simulink library "thc"  (R2021b)
settings: Solver=VariableStepAuto  StartTime=0.0  StopTime=10.0  RelTol=1e-3
undefined symbols (not defined in the file): ATHC_APTCQA_X_C, ATHC_APTCQB_X_C, ATHC_dAy_X_C, ATHC_Qeq_X_kmh, ATHC_VbaseC_X_C, ATHC_VbaseC_Y_W, ATHC_VbaseD_X_C, ATHC_VbaseH_X_C, FALSE, KTHC_ACMaxMinT_sec, KTHC_aDeice_K, KTHC_AGSDefLv_K, KTHC_AGSLv1_K, KTHC_AGSLv2_K, KTHC_AGSLv3_K, KTHC_AGSLv4_K, KTHC_AGSLv5_K, KTHC_AirIntUpdateT_sec, KTHC_APTCOneZoneMax_W, KTHC_APTCPeriod_cnt, KTHC_APTCPWMEN_flg, KTHC_APTCQMaxC_W, KTHC_APTCQminC_W, KTHC_APTCQminD_W, KTHC_APTCQminRe1_W, KTHC_APTCQminRe_W, KTHC_APTCQoffT_cnt, KTHC_APTCQonT_cnt, KTHC_APTCRiLeMaxDff_W, KTHC_APTCRiLeMinDff_W, KTHC_BatCoolT_cnt, KTHC_BatInTempDef_C, KTHC_bDeice_K, KTHC_CompMaxDeice_rpm, KTHC_CompMinDeice_rpm, KTHC_CompSotxvOp_K, KTHC_CompSotxvOpLow_rpm, KTHC_CompSpdmax_rpm, KTHC_CompSpdmaxBC1_rpm, KTHC_CompSpdmaxBC_rpm, KTHC_CompSpdmid1_rpm, KTHC_CompSpdmid2_rpm, KTHC_CompSpdmid3_rpm, KTHC_CompSpdmid_rpm, KTHC_CompSpdmin_rpm, KTHC_DAPTCQ1_W, KTHC_DAPTCQ2_W, KTHC_DAPTCQ3_W, KTHC_DcChSetTemp_C, KTHC_DehumidityEN_flg, KTHC_DeiceCycTime_K, KTHC_DriveLevelWPTCBAH1_W, KTHC_DriveLevelWPTCBAH2_W, KTHC_DriveLevelWPTCBAH3_W, KTHC_DriveLevelWPTCBAH4_W, KTHC_DriverSeatPos_flg, KTHC_DriveT1MinBAH_C, KTHC_DriveT2MaxBAH_C, KTHC_DriveT2MinBAH_C, KTHC_DriveT3MaxBAH_C ... (+379)
libraries: simulink x489
(part 16 of 17)

== stateflow chart thc/THC/ThermalControl/THCM_Conctrl/Thermal ==
  state OFF
    en:CabinMode=0;CompPID=0;CompSet=0;SOTXV=false;BlowerPID=0;APTCPID=0;EXV2PIDMode=0;ACSubMode=0;
    BattPump3=0;FrWPTCHeatPwr=0;BatteryMode=0;EDriveMode=uint8(0);EWP1=0;EWP2=0;AGS=0;TWV=100;ACMaxReq=false;
    ACD3Lv=0;BattPump3=0;FAN=0;FWV=false;
  state ON
    state WaterFill
      en:CabinMode=1;
      CompPID=0;
      CompSet=0;
      SOTXV=false;
      BlowerPID=0;
      APTCPID=0;
      EXV2PIDMode=0;
      ACSubMode=0;
      FrWPTCHeatPwr=0;
      BatteryMode=0;
      EDriveMode=uint8(0);
      AGS=0;
      TWV=35;
      ACMaxReq=false;
      ACD3Lv=0;
      FAN=0;
      FWV=false;
      state WF1
        en:EWP1=7;
        EWP2=7;
        BattPump3=7;
      state WF2
        en:EWP1=0;
        EWP2=0;
        BattPump3=0;
      (default) -> (junction 2447)
      (junction 2447) -> (junction 2449) [order 2]
      (junction 2447) -> WF1 [order 1] : [WaterFillReq==1]
      (junction 2449) -> WF2
    state Normal
      state Cabin [parallel]
        settings: executionOrder=2
        state ForceSWMode [parallel]
          settings: executionOrder=8
          state StandBy
            en:CabinModeReset=false;
          state Cooling
            du:CabinModeReset=false;
          state Heating
            du:CabinModeReset=false;
          (default) -> ON.Normal.Cabin.ForceSWMode.StandBy
          ON.Normal.Cabin.ForceSWMode.Cooling -> ON.Normal.Cabin.ForceSWMode.Cooling [order 3] : [Tamb<sigSetTempZon1StC&&....
              | TambMax-Tamb>KTHC_ForceLeaveCool_C]
              | {CabinModeReset=true;TambMax=Tamb;}
          ON.Normal.Cabin.ForceSWMode.StandBy -> ON.Normal.Cabin.ForceSWMode.Cooling [order 1] : [CabinMode==3]{TambMax=Tamb;}
          ON.Normal.Cabin.ForceSWMode.Cooling -> ON.Normal.Cabin.ForceSWMode.StandBy [order 1] : [CabinMode!=3]
          ON.Normal.Cabin.ForceSWMode.Cooling -> ON.Normal.Cabin.ForceSWMode.Cooling [order 2] : [Tamb>TambMax]{TambMax=Tamb;}
          ON.Normal.Cabin.ForceSWMode.Heating -> ON.Normal.Cabin.ForceSWMode.Heating [order 2] : [TambMin>Tamb]{TambMin=Tamb;}
          ON.Normal.Cabin.ForceSWMode.StandBy -> ON.Normal.Cabin.ForceSWMode.Heating [order 2] : [CabinMode==8||CabinMode==9]
              | {TambMin=Tamb;}
          ON.Normal.Cabin.ForceSWMode.Heating -> ON.Normal.Cabin.ForceSWMode.Heating [order 3] : [Tamb>sigSetTempZon1St&&....
              | Tamb-TambMin>KTHC_ForceLeaveHeat_C]
              | {CabinModeReset=true;TambMin=Tamb;}
          ON.Normal.Cabin.ForceSWMode.Heating -> ON.Normal.Cabin.ForceSWMode.StandBy [order 1] : [CabinMode!=8&&CabinMode!=9]
        state CabinCompReqCtrl [parallel]
          settings: executionOrder=1
          state Request
            en:CabinCompReq=true;
            ForceComp=false;
            du:ForceComp=false;
          state NoRequest
            en:CabinCompReq=false;
            CabinCompReqCancel=false;
            du:CabinCompReqCancel=false;
          (default) -> ON.Normal.Cabin.CabinCompReqCtrl.Request
          ON.Normal.Cabin.CabinCompReqCtrl.Request -> ON.Normal.Cabin.CabinCompReqCtrl.NoRequest : [(CompSpd<=KTHC_CompSpdmin_rpm&&Tincar<sigSetTempZon1StC-KTHC_DTcabin5_C)||....
              | CabinCompReqCancel]
          ON.Normal.Cabin.CabinCompReqCtrl.NoRequest -> ON.Normal.Cabin.CabinCompReqCtrl.Request : [Tincar>sigSetTempZon1StC+KTHC_DTreturn_C||ForceComp]
        state Main [parallel]
          settings: executionOrder=2
          state DeiceMode
            en:CabinMode=10;CompPID=9;CompSet=0;SOTXV=true;EXV2PIDMode=0;
            ex:CompSet=0;
            state CompSet [parallel]
              settings: executionOrder=2
              CompSet -> (junction 2150) : {CompSet=Bat_Out_Temp*KTHC_aDeice_K+KTHC_bDeice_K;}
              (junction 2150) -> (junction 2152) [order 1] : [CompSet<KTHC_CompMinDeice_rpm]{CompSet=KTHC_CompMinDeice_rpm;}
              (junction 2150) -> (junction 2154) [order 2]
              (junction 2154) -> (junction 2156) [order 1] : [CompSet>KTHC_CompMaxDeice_rpm]{CompSet=KTHC_CompMaxDeice_rpm;}
              (junction 2154) -> (junction 2158) [order 2]
            state ModeSelect [parallel]
              settings: executionOrder=1
              state DeiceMode1
                en:ACSubMode=1;
                APTCPID=0;
                BlowerPID=0;
              state DeiceMode2
                en:ACSubMode=2;
                APTCPID=6;
                BlowerPID=4;
              (default) -> (junction 2045)
              (junction 2045) -> DeiceMode1 [order 1] : [!AC]
              (junction 2045) -> DeiceMode2 [order 2]
              DeiceMode1 -> DeiceMode2 : [AC]
              DeiceMode2 -> DeiceMode1 : [!AC]
          state ACStandbyMode
            state Mode1
              en:CabinMode=1;
              CompPID=0;CompSet=0;
              SOTXV=false;
              BlowerPID=0;
              APTCPID=0;
              EXV2PIDMode=0;
              ACSubMode=0;
            state Mode2
              en:CabinMode=2;SOTXV=true;SOTXV=true;
              BlowerPID=0;
              APTCPID=0;
              EXV2PIDMode=0;
              state ACStandByMode
                en:ACSubMode=1;
                CompPID=2;
                CompSet=0;
              state ACStandByMode2
                en:ACSubMode=2;
                CompPID=3;
                CompSet=KTHC_CompSpdmaxBC_rpm;
              (default) -> ACStandByMode
              ACStandByMode -> ACStandByMode2 : [TBMax>KTHC_TBPmax_C]
              ACStandByMode2 -> ACStandByMode : [TBMax<KTHC_TBPmin_C]
            (junction 733) -> (junction 740)
            (junction 740) -> ON.Normal.Cabin.Main.ACStandbyMode.Mode1 [order 1] : [RequestCOMP==0]
            (junction 740) -> (junction 753) [order 2]
            ON.Normal.Cabin.Main.ACStandbyMode.Mode2 -> ON.Normal.Cabin.Main.ACStandbyMode.Mode1 : [RequestCOMP==0]
            ON.Normal.Cabin.Main.ACStandbyMode.Mode1 -> ON.Normal.Cabin.Main.ACStandbyMode.Mode2 : [RequestCOMP==1]
            (junction 753) -> ON.Normal.Cabin.Main.ACStandbyMode.Mode2
          state DCCharge
            en:CabinMode=11;
            APTCPID=9;
            CompSet=0;
            EXV2PIDMode=0;
            BlowerPID=0;
            state CompOFF
              ACSubMode=2;
              CompPID=0;
              SOTXV=true;
            state CompON
              en:ACSubMode=1;
              CompPID=11;
              SOTXV=false;
            (default) -> (junction 2495)
            (junction 2495) -> ON.Normal.Cabin.Main.DCCharge.CompON [order 2]
            (junction 2495) -> ON.Normal.Cabin.Main.DCCharge.CompOFF [order 1] : [Bat_In_Temp>KTHC_TWinmax_C]
            ON.Normal.Cabin.Main.DCCharge.CompON -> ON.Normal.Cabin.Main.DCCharge.CompOFF : [Bat_In_Temp>KTHC_TWinmax_C]
            ON.Normal.Cabin.Main.DCCharge.CompOFF -> ON.Normal.Cabin.Main.DCCharge.CompON : [after(600,tick)&&Bat_In_Temp<KTHC_TWinmin_C]
          state ACON
            state Cooling
              en:CabinMode=3;
              EXV2PIDMode=0;
              state ACCooling
                en:APTCPID=5;
                state Normal
                  state ACCoolingMode1and7
                    en:
                    CompPID=1;
                    CompSet=0;
                    SOTXV=false;
                    state ACCoolingMode1
                      en:BlowerPID=1;
                      ACSubMode=1;
                    state ACCoolingMode0
                      en:BlowerPID=0;
                      ACSubMode=0;
                    (default) -> (junction 2391)
                    (junction 2391) -> (junction 2393) [order 2]
                    (junction 2391) -> ACCoolingMode1 [order 1] : [FCool==0]
                    (junction 2393) -> ACCoolingMode0
                    ACCoolingMode0 -> ACCoolingMode1 : [FCool==0]
                    ACCoolingMode1 -> ACCoolingMode0 : [FCool>0]
                  state ACCoolingMode1_2
                    ex:APTCPID=5;
                    state Dehumidity
                      en:CabinMode=6;
                      ACSubMode=2;
                      CompPID=3;
                      BlowerPID=1;
                      SOTXV=false;
                      CompSet=KTHC_CompSpdmid3_rpm;
                      APTCPID=7;
                      ex:CabinMode=3;
                    state CompON
                      en:CabinMode=3;
                      APTCPID=8;
                      CompSet=0;
                      state ACCoolingMode6
                        en:
                        ACSubMode=6;
                        CompPID=10;
                        BlowerPID=0;
                        SOTXV=false;
                      state ACCoolingMode7
                        en:
                        ACSubMode=7;
                        CompPID=3;
                        BlowerPID=0;
                        SOTXV=true;
                      state ACCoolingMode2
                        en:
                        ACSubMode=2;
                        CompPID=10;
                        BlowerPID=1;
                        SOTXV=false;
                      (default) -> (junction 2413)
                      ON.Normal.Cabin.Main.ACON.Cooling.ACCooling.Normal.ACCoolingMode1_2.CompON -> (junction 2413) [order 1] : [hasChanged(FCool)]
                      (junction 2413) -> (junction 2420) [order 2]
                      (junction 2420) -> (junction 2431) [order 2]
                      (junction 2413) -> ACCoolingMode2 [order 1] : [FCool==0]
                      (junction 2420) -> ACCoolingMode6 [order 1] : [FCool==1]
                      (junction 2431) -> ACCoolingMode7
                    (default) -> (junction 2498)
                    (junction 2498) -> ON.Normal.Cabin.Main.ACON.Cooling.ACCooling.Normal.ACCoolingMode1_2.CompON [order 2]
                    (junction 2498) -> Dehumidity [order 1] : [Tincar<sigSetTempZon1StC-KTHC_DTcabin2_C&&....
                        | sigSetTempZon1St>17&&....
                        | (Tamb<KTHC_TambACmode7_C||....
                        | sigSetTempZon1StC>Tamb+KTHC_DTambsat4_C)]
                    Dehumidity -> ON.Normal.Cabin.Main.ACON.Cooling.ACCooling.Normal.ACCoolingMode1_2.CompON [order 2] : [(after(KTHC_DTimeCD1_K,tick)&&....
                        | Tincar>sigSetTempZon1StC+KTHC_DTcabin1_C)&&....
                        | (Tamb>KTHC_TambACmode6_C||....
                        | sigSetTempZon1StC<Tamb-KTHC_DTambsat3_C)||....
                        | sigSetTempZon1St<=17]
                    ON.Normal.Cabin.Main.ACON.Cooling.ACCooling.Normal.ACCoolingMode1_2.CompON -> Dehumidity [order 1] : [Tincar<sigSetTempZon1StC-KTHC_DTcabin2_C&&....
                        | sigSetTempZon1St>17&&....
                        | (Tamb<KTHC_TambACmode7_C||....
                        | sigSetTempZon1StC>Tamb+KTHC_DTambsat4_C)]
                  state ACCoolingMode1_3
                    en:ACSubMode=3;
                    CompPID=2;
                    CompSet=0;
                    BlowerPID=1;
                    SOTXV=!TincarPos;
                    du:SOTXV=!TincarPos;
                  ACCoolingMode1_2 -> ACCoolingMode1and7 [order 2] : [CabinCompReq]
                  (default) -> (junction 2360)
                  (junction 2360) -> ACCoolingMode1and7 [order 1] : [ACSubModeLAST == 1]
                  (junction 2360) -> ACCoolingMode1_2 [order 2] : [ACSubModeLAST == 2]
                  (junction 2360) -> (junction 2364) [order 3]
                  (junction 777) -> ACCoolingMode1_2 [order 1] : [RequestCOMP==0]
                  ACCoolingMode1_2 -> ACCoolingMode1_3 [order 1] : [RequestCOMP]
                  ACCoolingMode1_3 -> ACCoolingMode1_2 [order 2] : [!RequestCOMP]
                  ACCoolingMode1and7 -> (junction 777) [order 3] : [!CabinCompReq]
                  (junction 777) -> ACCoolingMode1_3 [order 2]
                  (junction 2364) -> ACCoolingMode1_3
                  ACCoolingMode1and7 -> ACCoolingMode1_3 [order 2] : [WaterCompReq]
                  ACCoolingMode1_3 -> ACCoolingMode1and7 [order 1] : [CabinCompReq&&....
                      | !WaterCompReq]
                state ACCoolingMode1_4
                  en:ACSubMode=4;CompPID=0;
                  CompSet=KTHC_CompSpdmaxBC1_rpm;BlowerPID=1;
                  SOTXV=!TincarPos;
                  du:SOTXV=!TincarPos;
                ACCoolingMode1_4 -> ACCoolingMode1_3 : [TBMax<KTHC_TBPmin_C]
                (junction 2357) -> ON.Normal.Cabin.Main.ACON.Cooling.ACCooling.Normal [order 2]
                ON.Normal.Cabin.Main.ACON.Cooling.ACCooling.Normal -> ACCoolingMode1_4 : [TBMax>KTHC_TBPmax_C]
                (junction 2357) -> ACCoolingMode1_4 [order 1] : [ACSubModeLAST == 4]
              state ACCoolingMode1_5
                en:
                BlowerPID=1;
                SOTXV=true;
                APTCPID=0;
                state CompMax
                  en:
                  CompPID=0;
                  CompSet=KTHC_CompSpdmaxBC1_rpm;
                state CompWin
                  en:
                  CompPID=2;
                  CompSet=0;
                state CompOFF
                  en:
                  CompPID=0;
                  CompSet=0;
                (junction 1698) -> (junction 1701) [order 2] : {ACSubMode=5;}
                (junction 1701) -> (junction 1705) [order 2]
                (junction 1698) -> CompMax [order 1] : [ACSubMode==4]{ACSubMode=5;}
                (junction 1701) -> CompWin [order 1] : [RequestCOMP]
                (junction 1705) -> ON.Normal.Cabin.Main.ACON.Cooling.ACCoolingMode1_5.CompOFF
                CompWin -> CompMax [order 1] : [TBMax>KTHC_TBPmax_C]
                CompWin -> ON.Normal.Cabin.Main.ACON.Cooling.ACCoolingMode1_5.CompOFF [order 2] : [!RequestCOMP]
                ON.Normal.Cabin.Main.ACON.Cooling.ACCoolingMode1_5.CompOFF -> CompWin : [RequestCOMP]
                CompMax -> CompWin : [TBMax<KTHC_TBPmin_C]
              (default) -> ACCoolingMode1and7
              ACCoolingMode1_5 -> (junction 2357) : [!EvapDefog]
              ACCooling -> (junction 1698) : [EvapDefog&&....
                  | Tamb>=KTHC_Trecymin_C]{ACSubModeLAST = ACSubMode;}
            state Duhumidity
              state DehumidityMode1and2
                state DehumidityMode1
                  en:CabinMode=4;ACSubMode=0;
                  CompPID=6;BlowerPID=3;
                  EXV2PIDMode=0;
                  APTCPID=5;SOTXV=false;
                state DehumidityMode2
                  en:CabinMode=5;
                  BlowerPID=3;
                  EXV2PIDMode=2;
                  SOTXV=false;
                  state DehumidityMode21
                    en:ACSubMode=1;
                    APTCPID=5;
                    CompPID=6;
                  state DehumidityMode22
                    en:ACSubMode=2;
                    APTCPID=2;
                    CompPID=8;
                  (default) -> DehumidityMode21
                  DehumidityMode21 -> DehumidityMode22 [order 1] : [after(100,tick)&&....
                      | (CompSpd>=KTHC_CompSpdmax_rpm||....
                      | ACHP>=KTHC_PhiDehum_kPa||....
                      | PT_High_T>=KTHC_ThiDehum_C)]
                  DehumidityMode22 -> DehumidityMode21 : [(after(KTHC_TimeD_K,tick)||....
                      | Tincar>sigSetTempZon1St+1)&&....
                      | APTCQ<=APTCQminD]
                DehumidityMode1and2 -> DehumidityMode22 [order 1] : [ErrCompForceOFF]
                (junction 1764) -> DehumidityMode1 [order 1] : [Tamb>KTHC_TambACmode2_C]
                (junction 1764) -> DehumidityMode2 [order 2] : [Tamb>KTHC_TambACmode3_C]
                DehumidityMode21 -> DehumidityMode1 [order 2] : [(CompSpd<=KTHC_CompSpdmin_rpm&&....
                    | Tincar>sigSetTempZon1St+KTHC_DTcabin3_C)||....
                    | (after(100,tick)&&....
                    | CompSpd<=KTHC_CompSpdmid1_rpm&&....
                    | Tincar>sigSetTempZon1St+KTHC_DTcabin12_C)]
                DehumidityMode1 -> DehumidityMode2 [order 2] : [CompSpd>KTHC_CompSpdmid_rpm||....
                    | ACHP>=KTHC_PhiDehum_kPa||....
                    | PT_High_T>KTHC_ThiDehum_C]
              state DehumidityMode4
                en:CabinMode=7;
                ACSubMode=0;
                CompPID=7;
                BlowerPID=3;
                EXV2PIDMode=0;
                SOTXV=true;
                APTCPID=4;
              state DehumidityMode3
                en:CabinMode=6;
                ACSubMode=1;
                CompPID=7;
                BlowerPID=3;
                EXV2PIDMode=0;
                SOTXV=false;
                APTCPID=3;
                FanMax=false;
                ex:ACD3Lv=0;
                state L2
                  en:ACD3Lv=2;
                state L3
                  en:ACD3Lv=3;
                state L4
                  en:ACD3Lv=4;
                state L5
                  en:ACD3Lv=5;
                  state Wait
                  state MAX
                    en:FanMax=true;
                  (default) -> ON.Normal.Cabin.Main.ACON.Duhumidity.DehumidityMode3.L5.Wait
                  ON.Normal.Cabin.Main.ACON.Duhumidity.DehumidityMode3.L5.Wait -> MAX : [after(150,tick)]
                (default) -> L2
                (junction 1803) -> L2 [order 1] : [Tincar<sigSetTempZon1St-1]
                L2 -> L3 : [Tincar>sigSetTempZon1St+1]
                L3 -> (junction 1803) : [after(150,tick)]
                (junction 1803) -> L4 [order 2] : [Tincar>sigSetTempZon1St+1]
                (junction 1808) -> L3 [order 1] : [Tincar<sigSetTempZon1St-1]
                L4 -> (junction 1808) : [after(150,tick)]
                (junction 1808) -> L5 [order 2] : [Tincar>sigSetTempZon1St+1]
                L5 -> L4 : [Tincar<sigSetTempZon1St-1]....
                    | {FanMax=false;}
              DehumidityMode3 -> DehumidityMode21 [order 1] : [!RequestCOMP]
              DehumidityMode1and2 -> DehumidityMode3 [order 3] : [RequestCOMP]
              DehumidityMode3 -> DehumidityMode4 [order 2] : [EvapDefog]
              DehumidityMode4 -> DehumidityMode3 [order 2] : [!EvapDefog]
            state HeatingMode
              en:ReqWasteHeatRecovery=true;SOTXV=true;
              ex:ReqWasteHeatRecovery=false;
              state HeatingMode1
                en:CabinMode=8;
                state HeatingMode11
                  en:CompPID=4;
                  APTCPID=5;
                  EXV2PIDMode=1;
                  ACSubMode=1;
                  BlowerPID=2;
                state HeatingMode12
                  en:CompPID=3;
                  APTCPID=5;
                  ACSubMode=2;
                  BlowerPID=2;
                  state EXV2ON
                    en:
                    EXV2PIDMode=1;
                    CompSet=KTHC_CompSpdmin_rpm;
                  state EXV2OFF
                    en:
                    EXV2PIDMode=0;
                    CompSet=0;
                  (default) -> EXV2ON
                  EXV2OFF -> EXV2ON : [Tincar<sigSetTempZon1St-KTHC_DTcabin9_C]
                  EXV2ON -> EXV2OFF : [Tincar>sigSetTempZon1St+KTHC_DTcabin9_C]
                HeatingMode11 -> HeatingMode12 [order 4] : [CompSpd<=KTHC_CompSpdmin_rpm&&....
                    | Tincar>sigSetTempZon1St+KTHC_DTcabin10_C]
                HeatingMode12 -> HeatingMode11 : [Tincar<sigSetTempZon1St-KTHC_DTreturn6_C]
              state HeatingMode2
                en:CabinMode=9;
                state HeatingMode21
                  en:CompPID=5;
                  APTCPID=1;
                  EXV2PIDMode=1;
                  ACSubMode=1;
                  BlowerPID=2;
                state APTCStart
                  en:CompPID=5;
                  APTCPID=1;
                  EXV2PIDMode=1;
                  BlowerPID=2;
                  ACSubMode=1;
                  state APTCStart
                  state APTCWait
                  (default) -> ON.Normal.Cabin.Main.ACON.HeatingMode.HeatingMode2.APTCStart.APTCStart
                  APTCWait -> ON.Normal.Cabin.Main.ACON.HeatingMode.HeatingMode2.APTCStart.APTCStart [order 1] : [APTCQ>KTHC_APTCQminRe1_W]
                  ON.Normal.Cabin.Main.ACON.HeatingMode.HeatingMode2.APTCStart.APTCStart -> APTCWait : [(!DfrstReq||Tincar>sigSetTempZon1St+KTHC_DTCabin11_C)&&....
                      | APTCQ<KTHC_APTCQminRe_W]{ACMaxReq=false;}
                state HeatingMode22
                  en:CompPID=0;
                  APTCPID=1;
                  EXV2PIDMode=0;
                  ACSubMode=2;
                  BlowerPID=2;
                  CompSet=0;
                HeatingMode21 -> ON.Normal.Cabin.Main.ACON.HeatingMode.HeatingMode2.APTCStart [order 1] : [APTCQ>=KTHC_APTCQminRe_W]
                ON.Normal.Cabin.Main.ACON.HeatingMode.HeatingMode2.APTCStart -> HeatingMode22 : [(EACProtectEnable==1||....
                    | PT_Low_P2<=KTHC_Plow2Setpoint_kPa)&&....
                    | CompSpd<=KTHC_CompSpdmin_rpm]
                (junction 2279) -> ON.Normal.Cabin.Main.ACON.HeatingMode.HeatingMode2.APTCStart : [(Motor_Out_Temp>KTHC_Twmset_C&&....
                    | PT_Low_P2>KTHC_Plow2Setpoint_kPa)||....
                    | Tamb>KTHC_Tambset_C]
                HeatingMode22 -> (junction 2279) : [after(3000,tick)]
              (default) -> (junction 972)
              (junction 972) -> (junction 973) [order 2]
              (junction 973) -> HeatingMode21
              (junction 972) -> HeatingMode11 [order 1] : [Tamb>KTHC_TambACmode4_C]
              HeatingMode11 -> HeatingMode21 [order 1] : [after(Timehu1,tick)&&Tincar<KTHC_DTh1_C]
              HeatingMode11 -> HeatingMode21 [order 2] : [after(Timehu2,tick)&&....
                  | (EACProtectEnable==1||CompSpd>=KTHC_CompSpdmax_rpm)&&Tincar<sigSetTempZon1St-KTHC_DTCabin11_C]
              HeatingMode11 -> HeatingMode21 [order 3] : [ACMaxReq||(DfrstReq&&Tincar<sigSetTempZon1St-KTHC_DTCabin11_C)]
              HeatingMode21 -> HeatingMode11 [order 2] : [after(KTHC_TimeRe2_sec*10,tick)&&Tincar>sigSetTempZon1St+KTHC_DTCabin11_C]
              APTCWait -> HeatingMode11 [order 2] : [after(KTHC_TimeRe1_sec*10,tick)]
            (junction 759) -> (junction 729)
            (junction 729) -> (junction 2287) [order 2]
            (junction 2287) -> (junction 724) [order 2]
            (junction 724) -> (junction 739) [order 2]
            (junction 729) -> ACCoolingMode1and7 [order 1] : [(!Tamb_Err&&(Tamb>KTHC_TambACmode1_C||(Tamb>KTHC_TambACmode3_C&&!KTHC_DehumidityEN_flg)))||(Tamb_Err&&Tincar>=sigSetTempZon1St)]
            (junction 2287) -> DehumidityMode1 [order 1] : [Tamb_Err]
            (junction 724) -> (junction 1764) [order 1] : [KTHC_DehumidityEN_flg]
            (junction 739) -> HeatingMode
            DehumidityMode1and2 -> ACCoolingMode1and7 [order 2] : [(!RequestCOMP&&Tincar>sigSetTempZon1StC+KTHC_DTcabin7_C&&....
                | sigSetTempZon1StC<Tamb-KTHC_DTambSat2_C)||....
                | Tincar>sigSetTempZon1StC+KTHC_DTreturn7_C||....
                | sigSetTempZon1St<=17]{ForceComp=true;}
            ACCoolingMode1and7 -> DehumidityMode1 [order 1] : [Tincar<sigSetTempZon1StC-KTHC_DTreturn1_C&&....
                | sigSetTempZon1StC>Tamb+KTHC_DTambSat1_C&&....
                | sigSetTempZon1St>17]
            DehumidityMode1 -> Dehumidity [order 1] : [(!RequestCOMP&&CompSpd<=KTHC_CompSpdmid2_rpm&&....
                | Tincar>sigSetTempZon1StC+KTHC_DTcabin4_C&&....
                | Tamb>KTHC_TambACmode5_C&&....
                | after(KTHC_DTimeCD2_K,tick))||....
                | (CompSpd<=KTHC_CompSpdmin_rpm&&....
                | ACHP>=KTHC_PhiDehum_kPa)]{CabinCompReqCancel=true;}...
            Dehumidity -> DehumidityMode1 [order 1] : [after(KTHC_DTimeCD_K,tick)&&...
                | KTHC_DehumidityEN_flg&&....
                | (Tincar<sigSetTempZon1StC-KTHC_DTreturn3_C||....
                | APTCQ>KTHC_APTCQMaxC_W)&&....
                | Tamb-sigSetTempZon1StC<KTHC_DTambSat_C]
            HeatingMode -> DehumidityMode22 [order 2] : [KTHC_DehumidityEN_flg&&...
                | !EvapDefog&&....
                | Tamb>KTHC_Tdeheat2_C]
            DehumidityMode1and2 -> HeatingMode21 [order 1] : [EvapDefog||Tamb<KTHC_Tdeheat1_C]
            DehumidityMode4 -> HeatingMode21 [order 1] : [!RequestCOMP]
            HeatingMode -> DehumidityMode4 [order 1] : [KTHC_DehumidityEN_flg&&RequestCOMP]
            DehumidityMode3 -> ACCoolingMode1_3 [order 3] : [FanMax&&Tincar>sigSetTempZon1St+KTHC_DTcabin6_C]
            ACCoolingMode1_3 -> DehumidityMode3 [order 3] : [KTHC_DehumidityEN_flg&&....
                | Tincar<sigSetTempZon1StC-KTHC_DTreturn2_C&&....
                | Tamb-sigSetTempZon1StC<KTHC_DTambSat_C]
            HeatingMode -> ON.Normal.Cabin.Main.ACON.Cooling [order 3] : [!KTHC_DehumidityEN_flg&&Tamb>=sigSetTempZon1St||....
                | (sigSetTempZon1St<=17&&Tamb>KTHC_TambSetLow_C)]
            ON.Normal.Cabin.Main.ACON.Cooling -> HeatingMode : [!KTHC_DehumidityEN_flg&&Tamb<sigSetTempZon1St]
          (default) -> (junction 761)
          (junction 761) -> (junction 733) [order 2]
          ACStandbyMode -> DeiceMode [order 2] : [DeiceModeReq==1]
          (junction 761) -> (junction 759) [order 1] : [(PwrSta>3&&AC)||....
              | (PwrSta>0&&PET)]
          ACON -> (junction 733) [order 2] : [(PwrSta<=3||!AC)&&....
              | (!PET||PwrSta==0)]
          (junction 2484) -> ON.Normal.Cabin.Main.ACStandbyMode.Mode1
          (junction 1972) -> (junction 2484) [order 2]
          DeiceMode -> (junction 1972) : [DeiceModeReq==0]
          ON.Normal.Cabin.Main.DCCharge -> (junction 2484) : [BatteryMode!=7]
          (junction 1972) -> (junction 973) [order 1] : [AC]
          ACON -> DeiceMode [order 3] : [DeiceModeReq==1]
          ACStandbyMode -> ON.Normal.Cabin.Main.DCCharge [order 3] : [BatteryMode==7]
          ACON -> ON.Normal.Cabin.Main.DCCharge [order 1] : [BatteryMode==7]
          ACStandbyMode -> (junction 729) [order 1] : [(PwrSta>3&&AC)||....
              | (PwrSta>0&&PET)]
          Main -> (junction 759) : [CabinModeReset]
        state WaterCompReqCtrl [parallel]
          settings: executionOrder=3
          state CoolingON
            note: 15 min
            state Request
              en:WaterCompReq=true;
            state ON
            state NoRequest
              en:WaterCompReq=false;
            ON.Normal.Cabin.WaterCompReqCtrl.CoolingON.ON -> (junction 1745) : [after(KTHC_Timewcd_K,tick)]
            (junction 1745) -> ON.Normal.Cabin.WaterCompReqCtrl.CoolingON.Request [order 1] : [RequestCOMP==1&&....
                | TBMax>=KTHC_T3MaxBC_C&&....
                | Bat_In_Temp>KTHC_T3winSetpointBC_C]....
            (junction 1745) -> (junction 1748) [order 2]
            ON.Normal.Cabin.WaterCompReqCtrl.CoolingON.Request -> ON.Normal.Cabin.WaterCompReqCtrl.CoolingON.NoRequest : [RequestCOMP==0||....
                | TBMax<KTHC_T4MinBC_C]
            ON.Normal.Cabin.WaterCompReqCtrl.CoolingON.NoRequest -> ON.Normal.Cabin.WaterCompReqCtrl.CoolingON.Request : [RequestCOMP==1&&....
                | TBMax>=KTHC_T3MaxBC_C&&....
                | Bat_In_Temp>KTHC_T3winSetpointBC_C]....
            (junction 1748) -> ON.Normal.Cabin.WaterCompReqCtrl.CoolingON.NoRequest
          state OFF
            en:WaterCompReq=false;
          (default) -> ON.Normal.Cabin.WaterCompReqCtrl.OFF
          ON.Normal.Cabin.WaterCompReqCtrl.OFF -> ON.Normal.Cabin.WaterCompReqCtrl.CoolingON.ON : [CabinMode==3]
          CoolingON -> ON.Normal.Cabin.WaterCompReqCtrl.OFF : [CabinMode!=3]
        state EvapDefogCtrl [parallel]
          settings: executionOrder=4
          state OFF
            en:EvapDefog=false;
          state ON
            en:EvapDefog=true;
          (default) -> ON.Normal.Cabin.EvapDefogCtrl.OFF
          ON.Normal.Cabin.EvapDefogCtrl.OFF -> ON.Normal.Cabin.EvapDefogCtrl.ON : [Tevap<Tice]
          ON.Normal.Cabin.EvapDefogCtrl.ON -> ON.Normal.Cabin.EvapDefogCtrl.OFF : [Tevap>Tdeice]
        state ACMaxReq [parallel]
          settings: executionOrder=6
          state OFF
            en:ACMaxReq=false;
          state ON
            en:ACMaxReq=true;
          (default) -> ON.Normal.Cabin.ACMaxReq.OFF
          ON.Normal.Cabin.ACMaxReq.OFF -> ON.Normal.Cabin.ACMaxReq.ON : [ACMax]
          ON.Normal.Cabin.ACMaxReq.ON -> ON.Normal.Cabin.ACMaxReq.OFF : [!ACMax]
        state ForceCool [parallel]
          settings: executionOrder=7
          state Normal
            en:FCool=0;
          state ForceCool
            state ForceCool2
              en:FCool=2;
            state ForceCool1
              en:FCool=1;
            (junction 2403) -> (junction 2408) [order 2] : [Tamb<KTHC_Trecymin_C]
            (junction 2403) -> ForceCool1 [order 1] : [Tamb>=KTHC_Trecymin_C]
            (junction 2408) -> ForceCool2
            ForceCool1 -> ForceCool2 : [Tamb<KTHC_Trecymin_C]
            ForceCool2 -> ForceCool1 : [Tamb>=KTHC_Trecymin_C]
          (default) -> ON.Normal.Cabin.ForceCool.Normal
          ON.Normal.Cabin.ForceCool.Normal -> (junction 2403) : [sigSetTempZon1St<=17&&....
              | Tamb<KTHC_Tcoolmin_C]
          ON.Normal.Cabin.ForceCool.ForceCool -> ON.Normal.Cabin.ForceCool.Normal : [sigSetTempZon1St>17||....
              | Tamb>=KTHC_Tcoolmin_C]
        state TincarPos [parallel]
          settings: executionOrder=5
          state Up
            TincarPos=true;
          state Down
            TincarPos=false;
          (default) -> (junction 1725)
          (junction 1725) -> Up [order 1] : [Tincar>sigSetTempZon1StC+KTHC_DTcabin_C]
          (junction 1725) -> (junction 1717) [order 2]
          Up -> Down : [Tincar<sigSetTempZon1StC-KTHC_DTcabin_C]
          Down -> Up : [Tincar>sigSetTempZon1StC+KTHC_DTcabin_C]
          (junction 1717) -> Down
      state Battery [parallel]
        settings: executionOrder=3
        state Battery [parallel]
          settings: executionOrder=3
          state Normal
            state Mode1
              en:BatteryMode=1;
              RequestCOMP=1;
              ex:RequestCOMP=0;
            state Mode2
              en:BatteryMode=2;
              FWV=true;
              ex:FWV=false;
            state Mode3
              en:BatteryMode=3;
            state Mode4
              en:BatteryMode=4;
              RequestTWV=1
              FWV=true;
              ex:RequestTWV=0;
              FWV=false;
            state Mode5
              en:BatteryMode=5;
            (default) -> (junction 600)
            (junction 600) -> ON.Normal.Battery.Battery.Normal.Mode1 [order 1] : [TBMax>KTHC_T1MaxBC_C]
            (junction 600) -> (junction 603) [order 2]
            ON.Normal.Battery.Battery.Normal.Mode1 -> ON.Normal.Battery.Battery.Normal.Mode2 [order 1] : [after(1200,tick)&&....
                | TBMin-Motor_In_Temp>KTHC_DTwBMoin1_C&&....
                | TBMax<KTHC_T4MinBC_C-1&&....
                | ChrgPlugSta<2]
            ON.Normal.Battery.Battery.Normal.Mode2 -> ON.Normal.Battery.Battery.Normal.Mode1 [order 2] : [TBMax>KTHC_T3MaxBC_C||....
                | (TBMin-Bat_In_Temp<KTHC_DTwBBin_C&&....
                | after(1200,tick))]
            (junction 601) -> ON.Normal.Battery.Battery.Normal.Mode1 [order 2]
            Mode3 -> ON.Normal.Battery.Battery.Normal.Mode1 [order 3] : [ChrgPlugSta==2&&....
                | TBMax>KTHC_TDcChgBC_C]
            ON.Normal.Battery.Battery.Normal.Mode1 -> Mode3 [order 2] : [(TBMax<KTHC_T2MinBC_C&&....
                | ChrgPlugSta<2)||....
                | (TBMax<KTHC_TDcChgBC_C-2&&....
                | ChrgPlugSta==2)]
            (junction 601) -> ON.Normal.Battery.Battery.Normal.Mode2 [order 1] : [TBMin-Motor_In_Temp>KTHC_DTwBMoin1_C]
            Mode3 -> (junction 601) [order 1] : [TBMax>KTHC_T1MaxBC_C&&....
                | ChrgPlugSta<2]
            ON.Normal.Battery.Battery.Normal.Mode2 -> Mode3 [order 1] : [TBMax<KTHC_T2MinBC_C]
            (junction 603) -> Mode3 [order 1] : [TBMin>=KTHC_T1MinBH_C]
            (junction 603) -> (junction 606) [order 2]
            Mode4 -> Mode3 [order 1] : [TBMin>KTHC_T2MaxBH_C||....
                | (ChrgPlugSta==0&&....
                | PreWPTC==0&&....
                | after(1200,tick)&&....
                | Bat_In_Temp-TBMax<=0&&....
                | TBMin>=KTHC_T2MinBH_C)]
            Mode3 -> (junction 604) [order 2] : [TBMin<KTHC_T1MinBH_C]
            Mode5 -> Mode3 [order 1] : [TBMin>KTHC_T2MaxBH_C||....
                | (ChrgPlugSta==0&&....
                | PreWPTC==0&&....
                | TBMin>=KTHC_T3MaxBH_C&&...
                | Motor_In_Temp-TBMax<=0)]
            (junction 604) -> Mode4 [order 2] : [Motor_In_Temp-TBMax>KTHC_DTwBMoin2_C]
            (junction 604) -> Mode5 [order 1] : [ChrgPlugSta>0||....
                | PreWPTC==1||....
                | TBMin<KTHC_T2MinBH_C]
            Mode4 -> Mode5 [order 2] : [((ChrgPlugSta>0||....
                | PreWPTC==1)&&....
                | TBMin<=KTHC_T2MaxBH_C)||....
                | (after(1200,tick)&&....
                | TBMin<KTHC_T2MinBH_C)]
            Mode5 -> Mode4 [order 2] : [ChrgPlugSta==0&&....
                | PreWPTC==0&&....
                | TBMin>=KTHC_T3MaxBH_C&&....
                | Motor_In_Temp-TBMax>KTHC_DTwBMoin3_C]
            (junction 606) -> Mode5
          state Deicing
            en:BatteryMode=6;
          note: BatteryMode
              | 0=OFF;
              | 1=Active Cooling;
              | 2=Passing Cooling;
              | 3=Isothermal Cycle;
              | 4=Passive Heating;
              | 5=Active Heating;
              | 6=Deicing;
          state BatteryDCChargeHeatingWoWPTC
            en:BatteryMode=7;
            BatDcCharge=true;
            ex:BatDcCharge=false;
            state Wait
            state FWVON
              en:FWV=true;
              ex:FWV=false;
            (default) -> ON.Normal.Battery.Battery.BatteryDCChargeHeatingWoWPTC.Wait
            ON.Normal.Battery.Battery.BatteryDCChargeHeatingWoWPTC.Wait -> FWVON : [after(50,tick)]
          state WaitForBalance
          (default) -> ON.Normal.Battery.Battery.Normal
          ON.Normal.Battery.Battery.Deicing -> (history) : [DeiceModeReq==0]
          ON.Normal.Battery.Battery.Normal -> ON.Normal.Battery.Battery.Deicing : [DeiceModeReq]
          WaitForBalance -> Mode3 : [after(50,tick)]
          BatteryDCChargeHeatingWoWPTC -> WaitForBalance : [!KTHC_WoWPTC_flg||....
              |  ChrgPlugSta!=2||....
              | TBMin>KTHC_T2MaxBH_C]
          Mode5 -> BatteryDCChargeHeatingWoWPTC [order 3] : [KTHC_WoWPTC_flg && ChrgPlugSta==2]
        state BattPump3 [parallel]
          settings: executionOrder=4
          state ON
            state OFF
              en:
              BattPump3=0;
              PumpONmode = 0;
            state Cooling
              en:
              PumpONmode = 1;
              state Level2
                en:BattPump3=2;
              state Level3
                en:BattPump3=3;
              state Level4
                en:BattPump3=4;
              state Level5
                en:BattPump3=5;
              (default) -> (junction 1568)
              (junction 1568) -> ON.Normal.Battery.BattPump3.ON.Cooling.Level2 [order 1] : [BattPump3<=2]
              (junction 1568) -> (junction 1570) [order 2]
              ON.Normal.Battery.BattPump3.ON.Cooling.Level2 -> ON.Normal.Battery.BattPump3.ON.Cooling.Level3 : [TBMax>KTHC_T2MaxBC_C]
              ON.Normal.Battery.BattPump3.ON.Cooling.Level3 -> ON.Normal.Battery.BattPump3.ON.Cooling.Level2 [order 2] : [TBMax<KTHC_T3MinBC_C]
              (junction 1570) -> ON.Normal.Battery.BattPump3.ON.Cooling.Level3 [order 1] : [BattPump3==3]
              (junction 1570) -> (junction 1573) [order 2]
              ON.Normal.Battery.BattPump3.ON.Cooling.Level3 -> ON.Normal.Battery.BattPump3.ON.Cooling.Level4 [order 1] : [TBMax>KTHC_T3MaxBC_C]
              ON.Normal.Battery.BattPump3.ON.Cooling.Level4 -> ON.Normal.Battery.BattPump3.ON.Cooling.Level3 [order 1] : [TBMax<KTHC_T4MinBC_C]
              (junction 1573) -> ON.Normal.Battery.BattPump3.ON.Cooling.Level4 [order 1] : [BattPump3==4]
              (junction 1573) -> (junction 1576) [order 2]
              ON.Normal.Battery.BattPump3.ON.Cooling.Level4 -> ON.Normal.Battery.BattPump3.ON.Cooling.Level5 [order 2] : [TBMax>KTHC_T4MaxBC_C]
              ON.Normal.Battery.BattPump3.ON.Cooling.Level5 -> ON.Normal.Battery.BattPump3.ON.Cooling.Level4 : [TBMax<KTHC_T5MinBC_C]
              (junction 1576) -> ON.Normal.Battery.BattPump3.ON.Cooling.Level5
            state IsothermalCycle
              en:
              PumpONmode = 2;
              state Level2
                en:BattPump3=1;
                state Higher3
                state Lower3
                (default) -> Higher3
                Lower3 -> Higher3 [order 1] : [TBMax-TBMin>3]
                Higher3 -> Lower3 : [TBMax-TBMin<=3]
              state Level4
                en:BattPump3=4;
              state Level3
                en:BattPump3=3;
              note: 5 min
              state Level1
                en:BattPump3=0;
              (default) -> (junction 674)
              (junction 673) -> (junction 674)
              (junction 674) -> (junction 675) [order 2]
              (junction 675) -> (junction 676) [order 2]
              (junction 676) -> (junction 2585) [order 1] : [TBMax-TBMin<2]
              (junction 677) -> (junction 673)
              (junction 674) -> ON.Normal.Battery.BattPump3.ON.IsothermalCycle.Level4 [order 1] : [TBMax-TBMin>=7]
              (junction 675) -> ON.Normal.Battery.BattPump3.ON.IsothermalCycle.Level3 [order 1] : [TBMax-TBMin>=5]
              (junction 676) -> ON.Normal.Battery.BattPump3.ON.IsothermalCycle.Level2 [order 2]
              (junction 2585) -> ON.Normal.Battery.BattPump3.ON.IsothermalCycle.Level1
              ON.Normal.Battery.BattPump3.ON.IsothermalCycle.Level4 -> (junction 678) : [TBMax-TBMin<7]
              ON.Normal.Battery.BattPump3.ON.IsothermalCycle.Level3 -> (junction 679) : [TBMax-TBMin>=7||....
                  | TBMax-TBMin<5]
              Lower3 -> ON.Normal.Battery.BattPump3.ON.IsothermalCycle.Level1 [order 2] : [after(KTHC_BatCoolT_cnt,tick)]
              Lower3 -> ON.Normal.Battery.BattPump3.ON.IsothermalCycle.Level1 [order 3] : [TBMax-TBMin<2]
              ON.Normal.Battery.BattPump3.ON.IsothermalCycle.Level1 -> (junction 681) : [TBMax-TBMin>3]
              ON.Normal.Battery.BattPump3.ON.IsothermalCycle.Level2 -> (junction 680) : [TBMax-TBMin>=5]
              (junction 681) -> (junction 680)
              (junction 678) -> (junction 677)
              (junction 679) -> (junction 678)
              (junction 680) -> (junction 679)
            state Heating
              en:
              PumpONmode = 3;
              state ActiveHeating
                ex:FrWPTCHeatPwr=0;
                state WPTC [parallel]
                  settings: executionOrder=2
                  state Level1
                    en:
                    FrWPTCHeatPwr=LevelWPTCBAH1;
                    du:
                    FrWPTCHeatPwr=LevelWPTCBAH1;
                  state Level2
                    en:
                    FrWPTCHeatPwr=LevelWPTCBAH2;
                    du:
                    FrWPTCHeatPwr=LevelWPTCBAH2;
                  state Level3
                    en:
                    FrWPTCHeatPwr=LevelWPTCBAH3;
                    du:
                    FrWPTCHeatPwr=LevelWPTCBAH3;
                  state Level4
                    en:
                    FrWPTCHeatPwr=LevelWPTCBAH4;
                    du:
                    FrWPTCHeatPwr=LevelWPTCBAH4;
                  (default) -> ON.Normal.Battery.BattPump3.ON.Heating.ActiveHeating.WPTC.Level1
                  ON.Normal.Battery.BattPump3.ON.Heating.ActiveHeating.WPTC.Level1 -> ON.Normal.Battery.BattPump3.ON.Heating.ActiveHeating.WPTC.Level2 : [after(30,tick)&&....
                      | Bat_In_Temp<KTHC_TWinmin_C]
                  ON.Normal.Battery.BattPump3.ON.Heating.ActiveHeating.WPTC.Level2 -> ON.Normal.Battery.BattPump3.ON.Heating.ActiveHeating.WPTC.Level1 [order 2] : [TBMin>T2MaxBAH||....
                      | (after(300,tick)&&Bat_In_Temp>KTHC_TWinmax_C)]
                  ON.Normal.Battery.BattPump3.ON.Heating.ActiveHeating.WPTC.Level2 -> ON.Normal.Battery.BattPump3.ON.Heating.ActiveHeating.WPTC.Level3 [order 1] : [TBMin<T2MinBAH&&....
                      | Bat_In_Temp<KTHC_TWinmin_C]
                  ON.Normal.Battery.BattPump3.ON.Heating.ActiveHeating.WPTC.Level3 -> ON.Normal.Battery.BattPump3.ON.Heating.ActiveHeating.WPTC.Level2 [order 2] : [TBMin>T3MaxBAH||....
                      | (after(300,tick)&&Bat_In_Temp>KTHC_TWinmax_C)]
                  ON.Normal.Battery.BattPump3.ON.Heating.ActiveHeating.WPTC.Level3 -> ON.Normal.Battery.BattPump3.ON.Heating.ActiveHeating.WPTC.Level4 [order 1] : [TBMin<T3MinBAH&&....
                      | Bat_In_Temp<KTHC_TWinmin_C]
                  ON.Normal.Battery.BattPump3.ON.Heating.ActiveHeating.WPTC.Level4 -> ON.Normal.Battery.BattPump3.ON.Heating.ActiveHeating.WPTC.Level3 : [TBMin>T4MaxBAH||....
                      | Bat_In_Temp>KTHC_TWinmax_C]
                state EWP_3 [parallel]
                  settings: executionOrder=1
                  state Level3
                    en:BattPump3=3;
                  state Level4
                    en:BattPump3=4;
                  state Level5
                    en:BattPump3=5;
                  (default) -> (junction 1590)
                  (junction 1590) -> ON.Normal.Battery.BattPump3.ON.Heating.ActiveHeating.EWP_3.Level3 [order 1] : [BattPump3<=3]
                  (junction 1590) -> (junction 1592) [order 2]
                  ON.Normal.Battery.BattPump3.ON.Heating.ActiveHeating.EWP_3.Level3 -> ON.Normal.Battery.BattPump3.ON.Heating.ActiveHeating.EWP_3.Level4 : [TBMin<T2MinBAH]
                  ON.Normal.Battery.BattPump3.ON.Heating.ActiveHeating.EWP_3.Level4 -> ON.Normal.Battery.BattPump3.ON.Heating.ActiveHeating.EWP_3.Level3 [order 2] : [TBMin>T3MaxBAH]
                  (junction 1592) -> ON.Normal.Battery.BattPump3.ON.Heating.ActiveHeating.EWP_3.Level4 [order 1] : [BattPump3==4]
                  (junction 1592) -> (junction 1595) [order 2]
                  ON.Normal.Battery.BattPump3.ON.Heating.ActiveHeating.EWP_3.Level4 -> ON.Normal.Battery.BattPump3.ON.Heating.ActiveHeating.EWP_3.Level5 [order 1] : [TBMin<T3MinBAH]
                  ON.Normal.Battery.BattPump3.ON.Heating.ActiveHeating.EWP_3.Level5 -> ON.Normal.Battery.BattPump3.ON.Heating.ActiveHeating.EWP_3.Level4 : [TBMin>T4MaxBAH]
                  (junction 1595) -> ON.Normal.Battery.BattPump3.ON.Heating.ActiveHeating.EWP_3.Level5
              state PassiveHeating
                state Level2
                  en:BattPump3=2;
                state Level3
                  en:BattPump3=3;
                state Level4
                  en:BattPump3=4;
                state Level5
                  en:BattPump3=5;
                (default) -> (junction 1579)
                (junction 1579) -> ON.Normal.Battery.BattPump3.ON.Heating.PassiveHeating.Level2 [order 1] : [BattPump3<=2]
                (junction 1579) -> (junction 1581) [order 2]
                ON.Normal.Battery.BattPump3.ON.Heating.PassiveHeating.Level2 -> ON.Normal.Battery.BattPump3.ON.Heating.PassiveHeating.Level3 : [TBMin<KTHC_T2MinBH_C]
                ON.Normal.Battery.BattPump3.ON.Heating.PassiveHeating.Level3 -> ON.Normal.Battery.BattPump3.ON.Heating.PassiveHeating.Level2 [order 2] : [TBMin>KTHC_T3MaxBH_C]
                (junction 1581) -> ON.Normal.Battery.BattPump3.ON.Heating.PassiveHeating.Level3 [order 1] : [BattPump3==3]
                (junction 1581) -> (junction 1584) [order 2]
                ON.Normal.Battery.BattPump3.ON.Heating.PassiveHeating.Level3 -> ON.Normal.Battery.BattPump3.ON.Heating.PassiveHeating.Level4 [order 1] : [TBMin<KTHC_T3MinBH_C]
                ON.Normal.Battery.BattPump3.ON.Heating.PassiveHeating.Level4 -> ON.Normal.Battery.BattPump3.ON.Heating.PassiveHeating.Level3 [order 1] : [TBMin>KTHC_T4MaxBH_C]
                (junction 1584) -> ON.Normal.Battery.BattPump3.ON.Heating.PassiveHeating.Level4 [order 1] : [BattPump3==4]
                (junction 1584) -> (junction 1587) [order 2]
                ON.Normal.Battery.BattPump3.ON.Heating.PassiveHeating.Level4 -> ON.Normal.Battery.BattPump3.ON.Heating.PassiveHeating.Level5 [order 2] : [TBMin<KTHC_T4MinBH_C]
                ON.Normal.Battery.BattPump3.ON.Heating.PassiveHeating.Level5 -> ON.Normal.Battery.BattPump3.ON.Heating.PassiveHeating.Level4 : [TBMin>KTHC_T5MaxBH_C]
                (junction 1587) -> ON.Normal.Battery.BattPump3.ON.Heating.PassiveHeating.Level5
              (default) -> (junction 1518)
              (junction 1518) -> PassiveHeating [order 1] : [BatteryMode==4]
              (junction 1518) -> ActiveHeating [order 2]
              PassiveHeating -> ActiveHeating : [BatteryMode==5]
              ActiveHeating -> PassiveHeating : [BatteryMode==4]
            ON.Normal.Battery.BattPump3.ON.OFF -> (junction 2115) : [BatteryMode>0&&BatteryMode<6]
            (junction 2115) -> (junction 643)
            (junction 645) -> ON.Normal.Battery.BattPump3.ON.OFF [order 2]
            (junction 643) -> (junction 644) [order 2]
            (junction 644) -> (junction 645) [order 2]
            (junction 643) -> ON.Normal.Battery.BattPump3.ON.Cooling [order 1] : [BatteryMode==1||....
                | BatteryMode==2]
            (junction 644) -> IsothermalCycle [order 1] : [BatteryMode==3]
            (junction 645) -> ON.Normal.Battery.BattPump3.ON.Heating [order 1] : [BatteryMode==4||....
                | BatteryMode==5]
            (junction 2367) -> ON.Normal.Battery.BattPump3.ON.OFF [order 1] : [PumpONmode == 0]
            ON.Normal.Battery.BattPump3.ON.Heating -> IsothermalCycle [order 1] : [BatteryMode==3]
            ON.Normal.Battery.BattPump3.ON.Cooling -> IsothermalCycle [order 1] : [BatteryMode==3]
            IsothermalCycle -> ON.Normal.Battery.BattPump3.ON.Heating [order 2] : [BatteryMode==4||....
                | BatteryMode==5]
            IsothermalCycle -> ON.Normal.Battery.BattPump3.ON.Cooling [order 1] : [BatteryMode==1||....
                | BatteryMode==2]
            (junction 2373) -> IsothermalCycle [order 2] : [PumpONmode == 2]
            ON.Normal.Battery.BattPump3.ON.Cooling -> ON.Normal.Battery.BattPump3.ON.Heating [order 2] : [BatteryMode==4||BatteryMode==5]
            ON.Normal.Battery.BattPump3.ON.Heating -> ON.Normal.Battery.BattPump3.ON.Cooling [order 2] : [BatteryMode==1||BatteryMode==2]
            (junction 2373) -> ON.Normal.Battery.BattPump3.ON.Cooling [order 1] : [PumpONmode == 1]
            (junction 2373) -> ON.Normal.Battery.BattPump3.ON.Heating [order 3]
            (junction 2375) -> (junction 2373)
            (junction 2367) -> (junction 2375) [order 2]
            (junction 2379) -> (junction 2367)
            (junction 2468) -> (junction 2379) : [BatteryMode<6]
          state Deicing
            en:BattPump3=6;
            ex:FrWPTCHeatPwr=0;
            state WPTC
              state Level1
                en:
                FrWPTCHeatPwr=LevelWPTCBAH1;
                du:
                FrWPTCHeatPwr=LevelWPTCBAH1;
              state Level2
                en:
                FrWPTCHeatPwr=LevelWPTCBAH2;
                du:
                FrWPTCHeatPwr=LevelWPTCBAH2;
              state Level3
                en:
                FrWPTCHeatPwr=LevelWPTCBAH3;
                du:
                FrWPTCHeatPwr=LevelWPTCBAH3;
              state Level4
                en:
                FrWPTCHeatPwr=LevelWPTCBAH4;
                du:
                FrWPTCHeatPwr=LevelWPTCBAH4;
              (default) -> ON.Normal.Battery.BattPump3.Deicing.WPTC.Level1
              ON.Normal.Battery.BattPump3.Deicing.WPTC.Level1 -> ON.Normal.Battery.BattPump3.Deicing.WPTC.Level2 : [TBMin<T1MinBAH&&....
                  | Bat_In_Temp<KTHC_TWinmin_C]
              ON.Normal.Battery.BattPump3.Deicing.WPTC.Level2 -> ON.Normal.Battery.BattPump3.Deicing.WPTC.Level1 [order 2] : [TBMin>T2MaxBAH||....
                  | (after(KTHC_Time0_K,tick)&&Bat_In_Temp>KTHC_TWinmax_C)]
              ON.Normal.Battery.BattPump3.Deicing.WPTC.Level2 -> ON.Normal.Battery.BattPump3.Deicing.WPTC.Level3 [order 1] : [TBMin<T2MinBAH&&....
                  | Bat_In_Temp<KTHC_TWinmin_C]
              ON.Normal.Battery.BattPump3.Deicing.WPTC.Level3 -> ON.Normal.Battery.BattPump3.Deicing.WPTC.Level2 [order 2] : [TBMin>T3MaxBAH||....
                  | (after(KTHC_Time0_K,tick)&&Bat_In_Temp>KTHC_TWinmax_C)]
              ON.Normal.Battery.BattPump3.Deicing.WPTC.Level3 -> ON.Normal.Battery.BattPump3.Deicing.WPTC.Level4 [order 1] : [TBMin<T3MinBAH&&....
                  | Bat_In_Temp<KTHC_TWinmin_C]
              ON.Normal.Battery.BattPump3.Deicing.WPTC.Level4 -> ON.Normal.Battery.BattPump3.Deicing.WPTC.Level3 : [TBMin>T4MaxBAH||....
                  | Bat_In_Temp>KTHC_TWinmax_C]
          state DCCharge
            en:BattPump3=8;
          (default) -> (junction 2115)
          ON.Normal.Battery.BattPump3.ON -> ON.Normal.Battery.BattPump3.Deicing [order 1] : [BatteryMode==6]
          ON.Normal.Battery.BattPump3.Deicing -> (junction 2468)
          ON.Normal.Battery.BattPump3.DCCharge -> (junction 2468)
          ON.Normal.Battery.BattPump3.ON -> ON.Normal.Battery.BattPump3.DCCharge [order 2] : [BatteryMode==7]
        state IVISWdet [parallel]
          settings: executionOrder=1
          state SWRelease
          state SWPress
          (default) -> (junction 2538)
          (junction 2538) -> SWRelease [order 1] : [!VINP_IVIWPTCSWSta_flg]
          (junction 2538) -> SWPress [order 2]
          SWPress -> SWRelease : [!VINP_IVIWPTCSWSta_flg]
          SWRelease -> SWPress : [VINP_IVIWPTCSWSta_flg]{PreWPTCModeCtrl.eWPTCSW}
        state PreWPTCModeCtrl [parallel]
          settings: executionOrder=2
          state StandBy
            en:VTHC_FDCTHCMPreWPTCHeatSta_enum=0;
            PreWPTC=0;
          state LowPower
            en:VTHC_FDCTHCMPreWPTCHeatSta_enum=2;
            PreWPTC=0;
          state ON
            en:VTHC_FDCTHCMPreWPTCHeatSta_enum=1;
            PreWPTC=1;
          (default) -> ON.Normal.Battery.PreWPTCModeCtrl.StandBy
          LowPower -> ON.Normal.Battery.PreWPTCModeCtrl.StandBy : [after(30,tick)]
          ON.Normal.Battery.PreWPTCModeCtrl.ON -> ON.Normal.Battery.PreWPTCModeCtrl.StandBy [order 2] : [(after(600,tick)&&BatteryMode!=5)||....
              | ChrgPlugSta>0]
          ON.Normal.Battery.PreWPTCModeCtrl.ON -> ON.Normal.Battery.PreWPTCModeCtrl.StandBy [order 1] : eWPTCSW
          ON.Normal.Battery.PreWPTCModeCtrl.StandBy -> ON.Normal.Battery.PreWPTCModeCtrl.ON : eWPTCSW[VINP_HVBattSOCDis_pct>=15]
          ON.Normal.Battery.PreWPTCModeCtrl.ON -> LowPower [order 3] : [VINP_HVBattSOCDis_pct<15]
      state EDrive [parallel]
        settings: executionOrder=4
        state EDriveMain [parallel]
          settings: executionOrder=3
          state NonCharging
            state Normal
              state Mode1
                en:
                EDriveMode=uint8(1);
                TWV=100;
                NormalMode = 1;
                state BatteryLevel [parallel]
                  settings: executionOrder=1
                  state LV1
                    en:BatteryLV=uint8(1);
                  state LV2
                    en:BatteryLV=uint8(2);
                  state LV3
                    en:BatteryLV=uint8(3);
                  state LV4
                    en:BatteryLV=uint8(4);
                  state LV5
                    en:BatteryLV=uint8(5);
                  (default) -> (junction 103)
                  (junction 103) -> ON.Normal.EDrive.EDriveMain.NonCharging.Normal.Mode1.BatteryLevel.LV1 [order 1] : [Tamb<25]
                  (junction 103) -> (junction 104) [order 2]
                  ON.Normal.EDrive.EDriveMain.NonCharging.Normal.Mode1.BatteryLevel.LV1 -> ON.Normal.EDrive.EDriveMain.NonCharging.Normal.Mode1.BatteryLevel.LV2 : [TBMax>KTHC_T1MaxBC_C]
                  ON.Normal.EDrive.EDriveMain.NonCharging.Normal.Mode1.BatteryLevel.LV2 -> ON.Normal.EDrive.EDriveMain.NonCharging.Normal.Mode1.BatteryLevel.LV1 [order 2] : [TBMax<KTHC_T2MinBC_C]
                  (junction 104) -> ON.Normal.EDrive.EDriveMain.NonCharging.Normal.Mode1.BatteryLevel.LV2 [order 1] : [Tamb<30]
                  (junction 104) -> (junction 105) [order 2]
                  ON.Normal.EDrive.EDriveMain.NonCharging.Normal.Mode1.BatteryLevel.LV2 -> ON.Normal.EDrive.EDriveMain.NonCharging.Normal.Mode1.BatteryLevel.LV3 [order 1] : [TBMax>KTHC_T2MaxBC_C]
                  ON.Normal.EDrive.EDriveMain.NonCharging.Normal.Mode1.BatteryLevel.LV3 -> ON.Normal.EDrive.EDriveMain.NonCharging.Normal.Mode1.BatteryLevel.LV2 [order 2] : [TBMax<KTHC_T3MinBC_C]
                  (junction 105) -> ON.Normal.EDrive.EDriveMain.NonCharging.Normal.Mode1.BatteryLevel.LV3 [order 1] : [Tamb<35]
                  (junction 105) -> (junction 106) [order 2]
                  ON.Normal.EDrive.EDriveMain.NonCharging.Normal.Mode1.BatteryLevel.LV3 -> ON.Normal.EDrive.EDriveMain.NonCharging.Normal.Mode1.BatteryLevel.LV4 [order 1] : [TBMax>KTHC_T3MaxBC_C]
                  ON.Normal.EDrive.EDriveMain.NonCharging.Normal.Mode1.BatteryLevel.LV4 -> ON.Normal.EDrive.EDriveMain.NonCharging.Normal.Mode1.BatteryLevel.LV3 [order 2] : [TBMax<KTHC_T4MinBC_C]
                  (junction 106) -> ON.Normal.EDrive.EDriveMain.NonCharging.Normal.Mode1.BatteryLevel.LV4 [order 1] : [Tamb<40]
                  (junction 106) -> (junction 107) [order 2]
                  ON.Normal.EDrive.EDriveMain.NonCharging.Normal.Mode1.BatteryLevel.LV4 -> ON.Normal.EDrive.EDriveMain.NonCharging.Normal.Mode1.BatteryLevel.LV5 [order 1] : [TBMax>KTHC_T4MaxBC_C]
                  ON.Normal.EDrive.EDriveMain.NonCharging.Normal.Mode1.BatteryLevel.LV5 -> ON.Normal.EDrive.EDriveMain.NonCharging.Normal.Mode1.BatteryLevel.LV4 : [TBMax<KTHC_T5MinBC_C]
                  (junction 107) -> ON.Normal.EDrive.EDriveMain.NonCharging.Normal.Mode1.BatteryLevel.LV5
                state DCDCLevel [parallel]
                  settings: executionOrder=3
                  state LV1
                    en:DCDCLV=uint8(1);
                  state LV2
                    en:DCDCLV=uint8(2);
                  state LV3
                    en:DCDCLV=uint8(3);
                  state LV4
                    en:DCDCLV=uint8(4);
                  state LV5
                    en:DCDCLV=uint8(5);
                  (default) -> (junction 11)
                  (junction 11) -> ON.Normal.EDrive.EDriveMain.NonCharging.Normal.Mode1.DCDCLevel.LV1 [order 1] : [Tamb<25]
                  (junction 11) -> (junction 12) [order 2]
                  ON.Normal.EDrive.EDriveMain.NonCharging.Normal.Mode1.DCDCLevel.LV1 -> ON.Normal.EDrive.EDriveMain.NonCharging.Normal.Mode1.DCDCLevel.LV2 : [Tdcdc>KTHC_T1MaxCCU_C]
                  ON.Normal.EDrive.EDriveMain.NonCharging.Normal.Mode1.DCDCLevel.LV2 -> ON.Normal.EDrive.EDriveMain.NonCharging.Normal.Mode1.DCDCLevel.LV1 [order 2] : [Tdcdc<KTHC_T2MinCCU_C]
                  (junction 12) -> ON.Normal.EDrive.EDriveMain.NonCharging.Normal.Mode1.DCDCLevel.LV2 [order 1] : [Tamb<30]
                  (junction 12) -> (junction 13) [order 2]
                  ON.Normal.EDrive.EDriveMain.NonCharging.Normal.Mode1.DCDCLevel.LV2 -> ON.Normal.EDrive.EDriveMain.NonCharging.Normal.Mode1.DCDCLevel.LV3 [order 1] : [Tdcdc>KTHC_T2MaxCCU_C]
                  ON.Normal.EDrive.EDriveMain.NonCharging.Normal.Mode1.DCDCLevel.LV3 -> ON.Normal.EDrive.EDriveMain.NonCharging.Normal.Mode1.DCDCLevel.LV2 [order 2] : [Tdcdc<KTHC_T3MinCCU_C]
                  (junction 13) -> ON.Normal.EDrive.EDriveMain.NonCharging.Normal.Mode1.DCDCLevel.LV3 [order 1] : [Tamb<35]
                  (junction 13) -> (junction 14) [order 2]
                  ON.Normal.EDrive.EDriveMain.NonCharging.Normal.Mode1.DCDCLevel.LV3 -> ON.Normal.EDrive.EDriveMain.NonCharging.Normal.Mode1.DCDCLevel.LV4 [order 1] : [Tdcdc>KTHC_T3MaxCCU_C]
                  ON.Normal.EDrive.EDriveMain.NonCharging.Normal.Mode1.DCDCLevel.LV4 -> ON.Normal.EDrive.EDriveMain.NonCharging.Normal.Mode1.DCDCLevel.LV3 [order 2] : [Tdcdc<KTHC_T4MinCCU_C]
                  (junction 14) -> ON.Normal.EDrive.EDriveMain.NonCharging.Normal.Mode1.DCDCLevel.LV4 [order 1] : [Tamb<40]
                  (junction 14) -> (junction 15) [order 2]
                  ON.Normal.EDrive.EDriveMain.NonCharging.Normal.Mode1.DCDCLevel.LV4 -> ON.Normal.EDrive.EDriveMain.NonCharging.Normal.Mode1.DCDCLevel.LV5 [order 1] : [Tdcdc>KTHC_T4MaxCCU_C]
                  ON.Normal.EDrive.EDriveMain.NonCharging.Normal.Mode1.DCDCLevel.LV5 -> ON.Normal.EDrive.EDriveMain.NonCharging.Normal.Mode1.DCDCLevel.LV4 : [Tdcdc<KTHC_T5MinCCU_C]
                  (junction 15) -> ON.Normal.EDrive.EDriveMain.NonCharging.Normal.Mode1.DCDCLevel.LV5
                state EWP1 [parallel]
                  settings: executionOrder=12
                  state S1
                    state Level5
                      en:EWP1=EDriveLV1;
                    (default) -> (junction 1663)
                    ON.Normal.EDrive.EDriveMain.NonCharging.Normal.Mode1.EWP1.S1 -> (junction 1663) [order 1] : [hasChanged(EDriveLV1)]
                    (junction 1663) -> ON.Normal.EDrive.EDriveMain.NonCharging.Normal.Mode1.EWP1.S1.Level5
                  state S2
                    state Level5
                      en:EWP1=EDriveLV2;
                    (default) -> (junction 1664)
                    ON.Normal.EDrive.EDriveMain.NonCharging.Normal.Mode1.EWP1.S2 -> (junction 1664) [order 1] : [hasChanged(EDriveLV2)]
                    (junction 1664) -> ON.Normal.EDrive.EDriveMain.NonCharging.Normal.Mode1.EWP1.S2.Level5
                  (default) -> (junction 1656)
                  (junction 1656) -> ON.Normal.EDrive.EDriveMain.NonCharging.Normal.Mode1.EWP1.S1 [order 1] : [BatteryMode==2]
                  (junction 1656) -> (junction 1650) [order 2]
                  ON.Normal.EDrive.EDriveMain.NonCharging.Normal.Mode1.EWP1.S1 -> ON.Normal.EDrive.EDriveMain.NonCharging.Normal.Mode1.EWP1.S2 [order 1] : [BatteryMode!=2]
                  ON.Normal.EDrive.EDriveMain.NonCharging.Normal.Mode1.EWP1.S2 -> ON.Normal.EDrive.EDriveMain.NonCharging.Normal.Mode1.EWP1.S1 [order 1] : [BatteryMode==2]
                  (junction 1650) -> ON.Normal.EDrive.EDriveMain.NonCharging.Normal.Mode1.EWP1.S2
                state OBCLevel [parallel]
                  settings: executionOrder=2
                  state LV1
                    en:OBCLV=uint8(1);
                  state LV2
                    en:OBCLV=uint8(2);
                  state LV3
                    en:OBCLV=uint8(3);
                  state LV4
                    en:OBCLV=uint8(4);
                  state LV5
                    en:OBCLV=uint8(5);
                  (default) -> (junction 164)
                  (junction 164) -> ON.Normal.EDrive.EDriveMain.NonCharging.Normal.Mode1.OBCLevel.LV1 [order 1] : [Tamb<25]
                  (junction 164) -> (junction 165) [order 2]
                  ON.Normal.EDrive.EDriveMain.NonCharging.Normal.Mode1.OBCLevel.LV1 -> ON.Normal.EDrive.EDriveMain.NonCharging.Normal.Mode1.OBCLevel.LV2 : [Tobc>KTHC_T1MaxCCU_C]
                  ON.Normal.EDrive.EDriveMain.NonCharging.Normal.Mode1.OBCLevel.LV2 -> ON.Normal.EDrive.EDriveMain.NonCharging.Normal.Mode1.OBCLevel.LV1 [order 2] : [Tobc<KTHC_T2MinCCU_C]
                  (junction 165) -> ON.Normal.EDrive.EDriveMain.NonCharging.Normal.Mode1.OBCLevel.LV2 [order 1] : [Tamb<30]
                  (junction 165) -> (junction 166) [order 2]
                  ON.Normal.EDrive.EDriveMain.NonCharging.Normal.Mode1.OBCLevel.LV2 -> ON.Normal.EDrive.EDriveMain.NonCharging.Normal.Mode1.OBCLevel.LV3 [order 1] : [Tobc>KTHC_T2MaxCCU_C]
                  ON.Normal.EDrive.EDriveMain.NonCharging.Normal.Mode1.OBCLevel.LV3 -> ON.Normal.EDrive.EDriveMain.NonCharging.Normal.Mode1.OBCLevel.LV2 [order 2] : [Tobc<KTHC_T3MinCCU_C]
                  (junction 166) -> ON.Normal.EDrive.EDriveMain.NonCharging.Normal.Mode1.OBCLevel.LV3 [order 1] : [Tamb<35]
                  (junction 166) -> (junction 167) [order 2]
                  ON.Normal.EDrive.EDriveMain.NonCharging.Normal.Mode1.OBCLevel.LV3 -> ON.Normal.EDrive.EDriveMain.NonCharging.Normal.Mode1.OBCLevel.LV4 [order 1] : [Tobc>KTHC_T3MaxCCU_C]
                  ON.Normal.EDrive.EDriveMain.NonCharging.Normal.Mode1.OBCLevel.LV4 -> ON.Normal.EDrive.EDriveMain.NonCharging.Normal.Mode1.OBCLevel.LV3 [order 2] : [Tobc<KTHC_T4MinCCU_C]
                  (junction 167) -> ON.Normal.EDrive.EDriveMain.NonCharging.Normal.Mode1.OBCLevel.LV4 [order 1] : [Tamb<40]
                  (junction 167) -> (junction 168) [order 2]
                  ON.Normal.EDrive.EDriveMain.NonCharging.Normal.Mode1.OBCLevel.LV4 -> ON.Normal.EDrive.EDriveMain.NonCharging.Normal.Mode1.OBCLevel.LV5 [order 1] : [Tobc>KTHC_T4MaxCCU_C]
                  ON.Normal.EDrive.EDriveMain.NonCharging.Normal.Mode1.OBCLevel.LV5 -> ON.Normal.EDrive.EDriveMain.NonCharging.Normal.Mode1.OBCLevel.LV4 : [Tobc<KTHC_T5MinCCU_C]
                  (junction 168) -> ON.Normal.EDrive.EDriveMain.NonCharging.Normal.Mode1.OBCLevel.LV5
                state EWP2 [parallel]
                  settings: executionOrder=15
                  state S1
                    state Level5
                      en:EWP2=EDriveLV1;
                    (default) -> (junction 1350)
                    ON.Normal.EDrive.EDriveMain.NonCharging.Normal.Mode1.EWP2.S1 -> (junction 1350) [order 1] : [hasChanged(EDriveLV1)]
                    (junction 1350) -> ON.Normal.EDrive.EDriveMain.NonCharging.Normal.Mode1.EWP2.S1.Level5
                  state S2
                    state Level5
                      en:EWP2=EDriveLV2;
                    (default) -> (junction 1372)
                    ON.Normal.EDrive.EDriveMain.NonCharging.Normal.Mode1.EWP2.S2 -> (junction 1372) [order 1] : [hasChanged(EDriveLV2)]
                    (junction 1372) -> ON.Normal.EDrive.EDriveMain.NonCharging.Normal.Mode1.EWP2.S2.Level5
                  (default) -> (junction 1341)
                  (junction 1341) -> ON.Normal.EDrive.EDriveMain.NonCharging.Normal.Mode1.EWP2.S1 [order 1] : [BatteryMode==2]
                  (junction 1341) -> (junction 1342) [order 2]
                  ON.Normal.EDrive.EDriveMain.NonCharging.Normal.Mode1.EWP2.S1 -> ON.Normal.EDrive.EDriveMain.NonCharging.Normal.Mode1.EWP2.S2 [order 1] : [BatteryMode!=2]
                  ON.Normal.EDrive.EDriveMain.NonCharging.Normal.Mode1.EWP2.S2 -> ON.Normal.EDrive.EDriveMain.NonCharging.Normal.Mode1.EWP2.S1 [order 1] : [BatteryMode==2]
                  (junction 1342) -> ON.Normal.EDrive.EDriveMain.NonCharging.Normal.Mode1.EWP2.S2
                state FrMCULevel [parallel]
                  settings: executionOrder=4
                  state LV1
                    en:FrMCULV=uint8(1);
                  state LV2
                    en:FrMCULV=uint8(2);
                  state LV3
                    en:FrMCULV=uint8(3);
                  state LV4
                    en:FrMCULV=uint8(4);
                  state LV5
                    en:FrMCULV=uint8(5);
                  (default) -> (junction 43)
                  (junction 43) -> ON.Normal.EDrive.EDriveMain.NonCharging.Normal.Mode1.FrMCULevel.LV1 [order 1] : [Tamb<25]
                  (junction 43) -> (junction 44) [order 2]
                  ON.Normal.EDrive.EDriveMain.NonCharging.Normal.Mode1.FrMCULevel.LV1 -> ON.Normal.EDrive.EDriveMain.NonCharging.Normal.Mode1.FrMCULevel.LV2 : [TFrMCU>KTHC_T1MaxMCU_C]
                  ON.Normal.EDrive.EDriveMain.NonCharging.Normal.Mode1.FrMCULevel.LV2 -> ON.Normal.EDrive.EDriveMain.NonCharging.Normal.Mode1.FrMCULevel.LV1 [order 2] : [TFrMCU<KTHC_T2MinMCU_C]
                  (junction 44) -> ON.Normal.EDrive.EDriveMain.NonCharging.Normal.Mode1.FrMCULevel.LV2 [order 1] : [Tamb<30]
                  (junction 44) -> (junction 45) [order 2]
                  ON.Normal.EDrive.EDriveMain.NonCharging.Normal.Mode1.FrMCULevel.LV2 -> ON.Normal.EDrive.EDriveMain.NonCharging.Normal.Mode1.FrMCULevel.LV3 [order 1] : [TFrMCU>KTHC_T2MaxMCU_C]
                  ON.Normal.EDrive.EDriveMain.NonCharging.Normal.Mode1.FrMCULevel.LV3 -> ON.Normal.EDrive.EDriveMain.NonCharging.Normal.Mode1.FrMCULevel.LV2 [order 2] : [TFrMCU<KTHC_T3MinMCU_C]
                  (junction 45) -> ON.Normal.EDrive.EDriveMain.NonCharging.Normal.Mode1.FrMCULevel.LV3 [order 1] : [Tamb<35]
                  (junction 45) -> (junction 46) [order 2]
                  ON.Normal.EDrive.EDriveMain.NonCharging.Normal.Mode1.FrMCULevel.LV3 -> ON.Normal.EDrive.EDriveMain.NonCharging.Normal.Mode1.FrMCULevel.LV4 [order 1] : [TFrMCU>KTHC_T3MaxMCU_C]
                  ON.Normal.EDrive.EDriveMain.NonCharging.Normal.Mode1.FrMCULevel.LV4 -> ON.Normal.EDrive.EDriveMain.NonCharging.Normal.Mode1.FrMCULevel.LV3 [order 2] : [TFrMCU<KTHC_T4MinMCU_C]
                  (junction 46) -> ON.Normal.EDrive.EDriveMain.NonCharging.Normal.Mode1.FrMCULevel.LV4 [order 1] : [Tamb<40]
                  (junction 46) -> (junction 47) [order 2]
                  ON.Normal.EDrive.EDriveMain.NonCharging.Normal.Mode1.FrMCULevel.LV4 -> ON.Normal.EDrive.EDriveMain.NonCharging.Normal.Mode1.FrMCULevel.LV5 [order 1] : [TFrMCU>KTHC_T4MaxMCU_C]
                  ON.Normal.EDrive.EDriveMain.NonCharging.Normal.Mode1.FrMCULevel.LV5 -> ON.Normal.EDrive.EDriveMain.NonCharging.Normal.Mode1.FrMCULevel.LV4 : [TFrMCU<KTHC_T5MinMCU_C]
                  (junction 47) -> ON.Normal.EDrive.EDriveMain.NonCharging.Normal.Mode1.FrMCULevel.LV5
                state AGS [parallel]
                  settings: executionOrder=13
                  state S0
                    en:AGS=0;
                  state S1
                    en:AGS=5;
                  state S2
                    en:AGS=max(EDriveLV1,3);
                  state S6
                    en:AGS=EDriveLV1;
                  state S3
                    en:AGS=max(EDriveLV4,ACD3Lv);
                  state S4
                    en:AGS=EDriveLV3;
                  state S5
                    en:AGS=EDriveLV4;
                  (default) -> (junction 1120)
                  ON.Normal.EDrive.EDriveMain.NonCharging.Normal.Mode1.AGS -> (junction 1120)
                  (junction 1120) -> S0 [order 1] : [Fags==3]
                  (junction 1120) -> (junction 215) [order 2]
                  (junction 215) -> ON.Normal.EDrive.EDriveMain.NonCharging.Normal.Mode1.AGS.S1 [order 1] : [Fags==1&&CabinMode!=6]
                  (junction 215) -> (junction 216) [order 2]
                  (junction 216) -> ON.Normal.EDrive.EDriveMain.NonCharging.Normal.Mode1.AGS.S2 [order 1] : [CabinMode==5]
                  (junction 216) -> (junction 1601) [order 2]
                  (junction 1601) -> ON.Normal.EDrive.EDriveMain.NonCharging.Normal.Mode1.AGS.S6 [order 1] : [CabinMode==4]
                  (junction 1601) -> (junction 217) [order 2]
                  (junction 217) -> ON.Normal.EDrive.EDriveMain.NonCharging.Normal.Mode1.AGS.S3 [order 1] : [CabinMode==6&&ACSubMode==1]
                  (junction 217) -> (junction 218) [order 2]
                  (junction 218) -> ON.Normal.EDrive.EDriveMain.NonCharging.Normal.Mode1.AGS.S4 [order 1] : [BatteryMode==2]
                  (junction 218) -> (junction 219) [order 2]
                  (junction 219) -> ON.Normal.EDrive.EDriveMain.NonCharging.Normal.Mode1.AGS.S5
                state RrLLCLevel [parallel]
                  settings: executionOrder=7
                  state LV1
                    en:RrLLCLV=uint8(1);
                  state LV2
                    en:RrLLCLV=uint8(2);
                  state LV3
                    en:RrLLCLV=uint8(3);
                  state LV4
                    en:RrLLCLV=uint8(4);
                  state LV5
                    en:RrLLCLV=uint8(5);
                  (default) -> (junction 2204)
                  (junction 2204) -> ON.Normal.EDrive.EDriveMain.NonCharging.Normal.Mode1.RrLLCLevel.LV1 [order 1] : [Tamb<25]
                  (junction 2204) -> (junction 2205) [order 2]
                  ON.Normal.EDrive.EDriveMain.NonCharging.Normal.Mode1.RrLLCLevel.LV1 -> ON.Normal.EDrive.EDriveMain.NonCharging.Normal.Mode1.RrLLCLevel.LV2 : [Rr_LLCTemp>KTHC_T1MaxLLC_C]
                  ON.Normal.EDrive.EDriveMain.NonCharging.Normal.Mode1.RrLLCLevel.LV2 -> ON.Normal.EDrive.EDriveMain.NonCharging.Normal.Mode1.RrLLCLevel.LV1 [order 2] : [Rr_LLCTemp<KTHC_T2MinLLC_C]
                  (junction 2205) -> ON.Normal.EDrive.EDriveMain.NonCharging.Normal.Mode1.RrLLCLevel.LV2 [order 1] : [Tamb<30]
                  (junction 2205) -> (junction 2206) [order 2]
                  ON.Normal.EDrive.EDriveMain.NonCharging.Normal.Mode1.RrLLCLevel.LV2 -> ON.Normal.EDrive.EDriveMain.NonCharging.Normal.Mode1.RrLLCLevel.LV3 [order 1] : [Rr_LLCTemp>KTHC_T2MaxLLC_C]
                  ON.Normal.EDrive.EDriveMain.NonCharging.Normal.Mode1.RrLLCLevel.LV3 -> ON.Normal.EDrive.EDriveMain.NonCharging.Normal.Mode1.RrLLCLevel.LV2 [order 2] : [Rr_LLCTemp<KTHC_T3MinLLC_C]
                  (junction 2206) -> ON.Normal.EDrive.EDriveMain.NonCharging.Normal.Mode1.RrLLCLevel.LV3 [order 1] : [Tamb<35]
                  (junction 2206) -> (junction 2207) [order 2]
                  ON.Normal.EDrive.EDriveMain.NonCharging.Normal.Mode1.RrLLCLevel.LV3 -> ON.Normal.EDrive.EDriveMain.NonCharging.Normal.Mode1.RrLLCLevel.LV4 [order 1] : [Rr_LLCTemp>KTHC_T3MaxLLC_C]
                  ON.Normal.EDrive.EDriveMain.NonCharging.Normal.Mode1.RrLLCLevel.LV4 -> ON.Normal.EDrive.EDriveMain.NonCharging.Normal.Mode1.RrLLCLevel.LV3 [order 2] : [Rr_LLCTemp<KTHC_T4MinLLC_C]
                  (junction 2207) -> ON.Normal.EDrive.EDriveMain.NonCharging.Normal.Mode1.RrLLCLevel.LV4 [order 1] : [Tamb<40]
                  (junction 2207) -> (junction 2208) [order 2]
                  ON.Normal.EDrive.EDriveMain.NonCharging.Normal.Mode1.RrLLCLevel.LV4 -> ON.Normal.EDrive.EDriveMain.NonCharging.Normal.Mode1.RrLLCLevel.LV5 [order 1] : [Rr_LLCTemp>KTHC_T4MaxLLC_C]
                  ON.Normal.EDrive.EDriveMain.NonCharging.Normal.Mode1.RrLLCLevel.LV5 -> ON.Normal.EDrive.EDriveMain.NonCharging.Normal.Mode1.RrLLCLevel.LV4 : [Rr_LLCTemp<KTHC_T5MinLLC_C]
                  (junction 2208) -> ON.Normal.EDrive.EDriveMain.NonCharging.Normal.Mode1.RrLLCLevel.LV5
                state RrMCULevel [parallel]
                  settings: executionOrder=5
                  state LV1
                    en:RrMCULV=uint8(1);
                  state LV2
                    en:RrMCULV=uint8(2);
                  state LV3
                    en:RrMCULV=uint8(3);
                  state LV4
                    en:RrMCULV=uint8(4);
                  state LV5
                    en:RrMCULV=uint8(5);
                  (default) -> (junction 132)
                  (junction 132) -> ON.Normal.EDrive.EDriveMain.NonCharging.Normal.Mode1.RrMCULevel.LV1 [order 1] : [Tamb<25]
                  (junction 132) -> (junction 133) [order 2]
                  ON.Normal.EDrive.EDriveMain.NonCharging.Normal.Mode1.RrMCULevel.LV1 -> ON.Normal.EDrive.EDriveMain.NonCharging.Normal.Mode1.RrMCULevel.LV2 : [TRrMCU>KTHC_T1MaxMCU_C]
                  ON.Normal.EDrive.EDriveMain.NonCharging.Normal.Mode1.RrMCULevel.LV2 -> ON.Normal.EDrive.EDriveMain.NonCharging.Normal.Mode1.RrMCULevel.LV1 [order 2] : [TRrMCU<KTHC_T2MinMCU_C]
                  (junction 133) -> ON.Normal.EDrive.EDriveMain.NonCharging.Normal.Mode1.RrMCULevel.LV2 [order 1] : [Tamb<30]
                  (junction 133) -> (junction 134) [order 2]
                  ON.Normal.EDrive.EDriveMain.NonCharging.Normal.Mode1.RrMCULevel.LV2 -> ON.Normal.EDrive.EDriveMain.NonCharging.Normal.Mode1.RrMCULevel.LV3 [order 1] : [TRrMCU>KTHC_T2MaxMCU_C]
                  ON.Normal.EDrive.EDriveMain.NonCharging.Normal.Mode1.RrMCULevel.LV3 -> ON.Normal.EDrive.EDriveMain.NonCharging.Normal.Mode1.RrMCULevel.LV2 [order 2] : [TRrMCU<KTHC_T3MinMCU_C]
                  (junction 134) -> ON.Normal.EDrive.EDriveMain.NonCharging.Normal.Mode1.RrMCULevel.LV3 [order 1] : [Tamb<35]
                  (junction 134) -> (junction 135) [order 2]
                  ON.Normal.EDrive.EDriveMain.NonCharging.Normal.Mode1.RrMCULevel.LV3 -> ON.Normal.EDrive.EDriveMain.NonCharging.Normal.Mode1.RrMCULevel.LV4 [order 1] : [TRrMCU>KTHC_T3MaxMCU_C]
                  ON.Normal.EDrive.EDriveMain.NonCharging.Normal.Mode1.RrMCULevel.LV4 -> ON.Normal.EDrive.EDriveMain.NonCharging.Normal.Mode1.RrMCULevel.LV3 [order 2] : [TRrMCU<KTHC_T4MinMCU_C]
                  (junction 135) -> ON.Normal.EDrive.EDriveMain.NonCharging.Normal.Mode1.RrMCULevel.LV4 [order 1] : [Tamb<40]
                  (junction 135) -> (junction 136) [order 2]
                  ON.Normal.EDrive.EDriveMain.NonCharging.Normal.Mode1.RrMCULevel.LV4 -> ON.Normal.EDrive.EDriveMain.NonCharging.Normal.Mode1.RrMCULevel.LV5 [order 1] : [TRrMCU>KTHC_T4MaxMCU_C]
                  ON.Normal.EDrive.EDriveMain.NonCharging.Normal.Mode1.RrMCULevel.LV5 -> ON.Normal.EDrive.EDriveMain.NonCharging.Normal.Mode1.RrMCULevel.LV4 : [TRrMCU<KTHC_T5MinMCU_C]
                  (junction 136) -> ON.Normal.EDrive.EDriveMain.NonCharging.Normal.Mode1.RrMCULevel.LV5
                state FAN [parallel]
                  settings: executionOrder=14
                  state S1
                    en:FAN=1;
                  state S2
                    en:FAN=max(EDriveLV1,3);
                  state S6
                    en:FAN=EDriveLV1;
                  state S3
                    en:FAN=max(EDriveLV4,ACD3Lv);
                  state S4
                    en:FAN=EDriveLV3;
                  state S5
                    en:FAN=EDriveLV4;
                  (default) -> (junction 1399)
                  ON.Normal.EDrive.EDriveMain.NonCharging.Normal.Mode1.FAN -> (junction 1399)
                  (junction 1399) -> ON.Normal.EDrive.EDriveMain.NonCharging.Normal.Mode1.FAN.S1 [order 1] : [Ffan==0]
                  (junction 1399) -> (junction 1403) [order 2]
                  (junction 1403) -> ON.Normal.EDrive.EDriveMain.NonCharging.Normal.Mode1.FAN.S2 [order 1] : [CabinMode==5]
                  (junction 1403) -> (junction 1646) [order 2]
                  (junction 1646) -> ON.Normal.EDrive.EDriveMain.NonCharging.Normal.Mode1.FAN.S6 [order 1] : [CabinMode==4]
                  (junction 1646) -> (junction 1428) [order 2]
                  (junction 1428) -> ON.Normal.EDrive.EDriveMain.NonCharging.Normal.Mode1.FAN.S3 [order 1] : [CabinMode==6&&ACSubMode==1]
                  (junction 1428) -> (junction 1473) [order 2]
                  (junction 1473) -> ON.Normal.EDrive.EDriveMain.NonCharging.Normal.Mode1.FAN.S4 [order 1] : [BatteryMode==2]
                  (junction 1473) -> (junction 1497) [order 2]
                  (junction 1497) -> ON.Normal.EDrive.EDriveMain.NonCharging.Normal.Mode1.FAN.S5
                state FrLLCLevel [parallel]
                  settings: executionOrder=8
                  state LV1
                    en:FrLLCLV=uint8(1);
                  state LV2
                    en:FrLLCLV=uint8(2);
                  state LV3
                    en:FrLLCLV=uint8(3);
                  state LV4
                    en:FrLLCLV=uint8(4);
                  state LV5
                    en:FrLLCLV=uint8(5);
                  (default) -> (junction 2233)
                  (junction 2233) -> ON.Normal.EDrive.EDriveMain.NonCharging.Normal.Mode1.FrLLCLevel.LV1 [order 1] : [Tamb<25]
                  (junction 2233) -> (junction 2234) [order 2]
                  ON.Normal.EDrive.EDriveMain.NonCharging.Normal.Mode1.FrLLCLevel.LV1 -> ON.Normal.EDrive.EDriveMain.NonCharging.Normal.Mode1.FrLLCLevel.LV2 : [Fr_LLCTemp>KTHC_T1MaxLLC_C]
                  ON.Normal.EDrive.EDriveMain.NonCharging.Normal.Mode1.FrLLCLevel.LV2 -> ON.Normal.EDrive.EDriveMain.NonCharging.Normal.Mode1.FrLLCLevel.LV1 [order 2] : [Fr_LLCTemp<KTHC_T2MinLLC_C]
                  (junction 2234) -> ON.Normal.EDrive.EDriveMain.NonCharging.Normal.Mode1.FrLLCLevel.LV2 [order 1] : [Tamb<30]
                  (junction 2234) -> (junction 2235) [order 2]
                  ON.Normal.EDrive.EDriveMain.NonCharging.Normal.Mode1.FrLLCLevel.LV2 -> ON.Normal.EDrive.EDriveMain.NonCharging.Normal.Mode1.FrLLCLevel.LV3 [order 1] : [Fr_LLCTemp>KTHC_T2MaxLLC_C]
                  ON.Normal.EDrive.EDriveMain.NonCharging.Normal.Mode1.FrLLCLevel.LV3 -> ON.Normal.EDrive.EDriveMain.NonCharging.Normal.Mode1.FrLLCLevel.LV2 [order 2] : [Fr_LLCTemp<KTHC_T3MinLLC_C]
                  (junction 2235) -> ON.Normal.EDrive.EDriveMain.NonCharging.Normal.Mode1.FrLLCLevel.LV3 [order 1] : [Tamb<35]
                  (junction 2235) -> (junction 2236) [order 2]
                  ON.Normal.EDrive.EDriveMain.NonCharging.Normal.Mode1.FrLLCLevel.LV3 -> ON.Normal.EDrive.EDriveMain.NonCharging.Normal.Mode1.FrLLCLevel.LV4 [order 1] : [Fr_LLCTemp>KTHC_T3MaxLLC_C]
                  ON.Normal.EDrive.EDriveMain.NonCharging.Normal.Mode1.FrLLCLevel.LV4 -> ON.Normal.EDrive.EDriveMain.NonCharging.Normal.Mode1.FrLLCLevel.LV3 [order 2] : [Fr_LLCTemp<KTHC_T4MinLLC_C]
                  (junction 2236) -> ON.Normal.EDrive.EDriveMain.NonCharging.Normal.Mode1.FrLLCLevel.LV4 [order 1] : [Tamb<40]
                  (junction 2236) -> (junction 2237) [order 2]
                  ON.Normal.EDrive.EDriveMain.NonCharging.Normal.Mode1.FrLLCLevel.LV4 -> ON.Normal.EDrive.EDriveMain.NonCharging.Normal.Mode1.FrLLCLevel.LV5 [order 1] : [Fr_LLCTemp>KTHC_T4MaxLLC_C]
                  ON.Normal.EDrive.EDriveMain.NonCharging.Normal.Mode1.FrLLCLevel.LV5 -> ON.Normal.EDrive.EDriveMain.NonCharging.Normal.Mode1.FrLLCLevel.LV4 : [Fr_LLCTemp<KTHC_T5MinLLC_C]
                  (junction 2237) -> ON.Normal.EDrive.EDriveMain.NonCharging.Normal.Mode1.FrLLCLevel.LV5
                state RrTMLevel [parallel]
                  settings: executionOrder=6
                  state LV1
                    en:RrTMLV=uint8(1);
                  state LV2
                    en:RrTMLV=uint8(2);
                  state LV3
                    en:RrTMLV=uint8(3);
                  state LV4
                    en:RrTMLV=uint8(4);
                  state LV5
                    en:RrTMLV=uint8(5);
                  (default) -> (junction 237)
                  (junction 237) -> ON.Normal.EDrive.EDriveMain.NonCharging.Normal.Mode1.RrTMLevel.LV1 [order 1] : [Tamb<25]
                  (junction 237) -> (junction 238) [order 2]
                  ON.Normal.EDrive.EDriveMain.NonCharging.Normal.Mode1.RrTMLevel.LV1 -> ON.Normal.EDrive.EDriveMain.NonCharging.Normal.Mode1.RrTMLevel.LV2 : [TRrTM>KTHC_T1MaxMT_C]
                  ON.Normal.EDrive.EDriveMain.NonCharging.Normal.Mode1.RrTMLevel.LV2 -> ON.Normal.EDrive.EDriveMain.NonCharging.Normal.Mode1.RrTMLevel.LV1 [order 2] : [TRrTM<KTHC_T2MinMT_C]
                  (junction 238) -> ON.Normal.EDrive.EDriveMain.NonCharging.Normal.Mode1.RrTMLevel.LV2 [order 1] : [Tamb<30]
                  (junction 238) -> (junction 239) [order 2]
                  ON.Normal.EDrive.EDriveMain.NonCharging.Normal.Mode1.RrTMLevel.LV2 -> ON.Normal.EDrive.EDriveMain.NonCharging.Normal.Mode1.RrTMLevel.LV3 [order 1] : [TRrTM>KTHC_T2MaxMT_C]
                  ON.Normal.EDrive.EDriveMain.NonCharging.Normal.Mode1.RrTMLevel.LV3 -> ON.Normal.EDrive.EDriveMain.NonCharging.Normal.Mode1.RrTMLevel.LV2 [order 2] : [TRrTM<KTHC_T3MinMT_C]
                  (junction 239) -> ON.Normal.EDrive.EDriveMain.NonCharging.Normal.Mode1.RrTMLevel.LV3 [order 1] : [Tamb<35]
                  (junction 239) -> (junction 240) [order 2]
                  ON.Normal.EDrive.EDriveMain.NonCharging.Normal.Mode1.RrTMLevel.LV3 -> ON.Normal.EDrive.EDriveMain.NonCharging.Normal.Mode1.RrTMLevel.LV4 [order 1] : [TRrTM>KTHC_T3MaxMT_C]
                  ON.Normal.EDrive.EDriveMain.NonCharging.Normal.Mode1.RrTMLevel.LV4 -> ON.Normal.EDrive.EDriveMain.NonCharging.Normal.Mode1.RrTMLevel.LV3 [order 2] : [TRrTM<KTHC_T4MinMT_C]
                  (junction 240) -> ON.Normal.EDrive.EDriveMain.NonCharging.Normal.Mode1.RrTMLevel.LV4 [order 1] : [Tamb<40]
                  (junction 240) -> (junction 241) [order 2]
                  ON.Normal.EDrive.EDriveMain.NonCharging.Normal.Mode1.RrTMLevel.LV4 -> ON.Normal.EDrive.EDriveMain.NonCharging.Normal.Mode1.RrTMLevel.LV5 [order 1] : [TRrTM>KTHC_T4MaxMT_C]
                  ON.Normal.EDrive.EDriveMain.NonCharging.Normal.Mode1.RrTMLevel.LV5 -> ON.Normal.EDrive.EDriveMain.NonCharging.Normal.Mode1.RrTMLevel.LV4 : [TRrTM<KTHC_T5MinMT_C]
                  (junction 241) -> ON.Normal.EDrive.EDriveMain.NonCharging.Normal.Mode1.RrTMLevel.LV5
                state FrTMLevel [parallel]
                  settings: executionOrder=9
                  state LV1
                    en:FrTMLV=uint8(1);
                  state LV2
                    en:FrTMLV=uint8(2);
                  state LV3
                    en:FrTMLV=uint8(3);
                  state LV4
                    en:FrTMLV=uint8(4);
                  state LV5
                    en:FrTMLV=uint8(5);
                  (default) -> (junction 297)
                  (junction 297) -> ON.Normal.EDrive.EDriveMain.NonCharging.Normal.Mode1.FrTMLevel.LV1 [order 1] : [Tamb<25]
                  (junction 297) -> (junction 298) [order 2]
                  ON.Normal.EDrive.EDriveMain.NonCharging.Normal.Mode1.FrTMLevel.LV1 -> ON.Normal.EDrive.EDriveMain.NonCharging.Normal.Mode1.FrTMLevel.LV2 : [TFrTM>KTHC_T1MaxMT_C]
                  ON.Normal.EDrive.EDriveMain.NonCharging.Normal.Mode1.FrTMLevel.LV2 -> ON.Normal.EDrive.EDriveMain.NonCharging.Normal.Mode1.FrTMLevel.LV1 [order 2] : [TFrTM<KTHC_T2MinMT_C]
                  (junction 298) -> ON.Normal.EDrive.EDriveMain.NonCharging.Normal.Mode1.FrTMLevel.LV2 [order 1] : [Tamb<30]
                  (junction 298) -> (junction 299) [order 2]
                  ON.Normal.EDrive.EDriveMain.NonCharging.Normal.Mode1.FrTMLevel.LV2 -> ON.Normal.EDrive.EDriveMain.NonCharging.Normal.Mode1.FrTMLevel.LV3 [order 1] : [TFrTM>KTHC_T2MaxMT_C]
                  ON.Normal.EDrive.EDriveMain.NonCharging.Normal.Mode1.FrTMLevel.LV3 -> ON.Normal.EDrive.EDriveMain.NonCharging.Normal.Mode1.FrTMLevel.LV2 [order 2] : [TFrTM<KTHC_T3MinMT_C]
                  (junction 299) -> ON.Normal.EDrive.EDriveMain.NonCharging.Normal.Mode1.FrTMLevel.LV3 [order 1] : [Tamb<35]
                  (junction 299) -> (junction 300) [order 2]
                  ON.Normal.EDrive.EDriveMain.NonCharging.Normal.Mode1.FrTMLevel.LV3 -> ON.Normal.EDrive.EDriveMain.NonCharging.Normal.Mode1.FrTMLevel.LV4 [order 1] : [TFrTM>KTHC_T3MaxMT_C]
                  ON.Normal.EDrive.EDriveMain.NonCharging.Normal.Mode1.FrTMLevel.LV4 -> ON.Normal.EDrive.EDriveMain.NonCharging.Normal.Mode1.FrTMLevel.LV3 [order 2] : [TFrTM<KTHC_T4MinMT_C]
                  (junction 300) -> ON.Normal.EDrive.EDriveMain.NonCharging.Normal.Mode1.FrTMLevel.LV4 [order 1] : [Tamb<40]
                  (junction 300) -> (junction 301) [order 2]
                  ON.Normal.EDrive.EDriveMain.NonCharging.Normal.Mode1.FrTMLevel.LV4 -> ON.Normal.EDrive.EDriveMain.NonCharging.Normal.Mode1.FrTMLevel.LV5 [order 1] : [TFrTM>KTHC_T4MaxMT_C]
                  ON.Normal.EDrive.EDriveMain.NonCharging.Normal.Mode1.FrTMLevel.LV5 -> ON.Normal.EDrive.EDriveMain.NonCharging.Normal.Mode1.FrTMLevel.LV4 : [TFrTM<KTHC_T5MinMT_C]
                  (junction 301) -> ON.Normal.EDrive.EDriveMain.NonCharging.Normal.Mode1.FrTMLevel.LV5
                state ACPressureHi [parallel]
                  settings: executionOrder=10
                  state LV1
                    en:ACHPLV=uint8(1);
                  state LV2
                    en:ACHPLV=uint8(2);
                  state LV3
                    en:ACHPLV=uint8(3);
                  state LV4
                    en:ACHPLV=uint8(4);
                  state LV5
                    en:ACHPLV=uint8(5);
                  (default) -> (junction 335)
                  (junction 335) -> ON.Normal.EDrive.EDriveMain.NonCharging.Normal.Mode1.ACPressureHi.LV1 [order 1] : [CabinMode<=1]
                  (junction 335) -> (junction 336) [order 2]
                  ON.Normal.EDrive.EDriveMain.NonCharging.Normal.Mode1.ACPressureHi.LV1 -> ON.Normal.EDrive.EDriveMain.NonCharging.Normal.Mode1.ACPressureHi.LV2 : [CabinMode>1]
                  ON.Normal.EDrive.EDriveMain.NonCharging.Normal.Mode1.ACPressureHi.LV2 -> ON.Normal.EDrive.EDriveMain.NonCharging.Normal.Mode1.ACPressureHi.LV1 [order 2] : [CabinMode<=1]
                  (junction 336) -> ON.Normal.EDrive.EDriveMain.NonCharging.Normal.Mode1.ACPressureHi.LV2 [order 1] : [CabinMode>1]
                  (junction 336) -> (junction 337) [order 2]
                  ON.Normal.EDrive.EDriveMain.NonCharging.Normal.Mode1.ACPressureHi.LV2 -> ON.Normal.EDrive.EDriveMain.NonCharging.Normal.Mode1.ACPressureHi.LV3 [order 1] : [ACHP>KTHC_P2MaxHi_kPa]
                  ON.Normal.EDrive.EDriveMain.NonCharging.Normal.Mode1.ACPressureHi.LV3 -> ON.Normal.EDrive.EDriveMain.NonCharging.Normal.Mode1.ACPressureHi.LV2 [order 2] : [ACHP<KTHC_P3MinHi_kPa]
                  (junction 337) -> ON.Normal.EDrive.EDriveMain.NonCharging.Normal.Mode1.ACPressureHi.LV3 [order 1] : [ACHP<KTHC_P4MinHi_kPa]
                  (junction 337) -> (junction 338) [order 2]
                  ON.Normal.EDrive.EDriveMain.NonCharging.Normal.Mode1.ACPressureHi.LV3 -> ON.Normal.EDrive.EDriveMain.NonCharging.Normal.Mode1.ACPressureHi.LV4 [order 1] : [ACHP>KTHC_P3MaxHi_kPa]
                  ON.Normal.EDrive.EDriveMain.NonCharging.Normal.Mode1.ACPressureHi.LV4 -> ON.Normal.EDrive.EDriveMain.NonCharging.Normal.Mode1.ACPressureHi.LV3 [order 2] : [ACHP<KTHC_P4MinHi_kPa]
                  (junction 338) -> ON.Normal.EDrive.EDriveMain.NonCharging.Normal.Mode1.ACPressureHi.LV4 [order 1] : [ACHP<KTHC_P5MinHi_kPa]
                  (junction 338) -> (junction 339) [order 2]
                  ON.Normal.EDrive.EDriveMain.NonCharging.Normal.Mode1.ACPressureHi.LV4 -> ON.Normal.EDrive.EDriveMain.NonCharging.Normal.Mode1.ACPressureHi.LV5 [order 1] : [ACHP>KTHC_P4MaxHi_kPa]
                  ON.Normal.EDrive.EDriveMain.NonCharging.Normal.Mode1.ACPressureHi.LV5 -> ON.Normal.EDrive.EDriveMain.NonCharging.Normal.Mode1.ACPressureHi.LV4 : [ACHP<KTHC_P5MinHi_kPa]
                  (junction 339) -> ON.Normal.EDrive.EDriveMain.NonCharging.Normal.Mode1.ACPressureHi.LV5
                state EDriveLevel [parallel]
                  settings: executionOrder=11
                  state STOP
                  (default) -> (junction 367)
                  EDriveLevel -> (junction 367)
                  (junction 367) -> STOP : {EDriveLV2=max(OBCLV,DCDCLV,FrMCULV,RrMCULV,FrTMLV,RrTMLV,FrLLCLV,RrLLCLV);....
                      | EDriveLV1=max(BatteryLV,EDriveLV2);....
                      | EDriveLV3=max(EDriveLV1,ACHPLV);...
                      | EDriveLV4=max(EDriveLV2,ACHPLV);}
              state Mode2
                en:
                EDriveMode=uint8(2);
                NormalMode = 2;
                state EWP1 [parallel]
                  settings: executionOrder=1
                  state Level4
                    en:EWP1=4;
                  state Level2
                    en:EWP1=2;
                  state Level3
                    en:EWP1=3;
                  (default) -> (junction 374)
                  (junction 374) -> ON.Normal.EDrive.EDriveMain.NonCharging.Normal.Mode2.EWP1.Level4 [order 1] : [PRC]
                  (junction 374) -> (junction 377) [order 2]
                  ON.Normal.EDrive.EDriveMain.NonCharging.Normal.Mode2.EWP1.Level4 -> (junction 375) : [!PRC]
                  ON.Normal.EDrive.EDriveMain.NonCharging.Normal.Mode2.EWP1.Level2 -> ON.Normal.EDrive.EDriveMain.NonCharging.Normal.Mode2.EWP1.Level4 [order 1] : [PRC]
                  ON.Normal.EDrive.EDriveMain.NonCharging.Normal.Mode2.EWP1.Level3 -> ON.Normal.EDrive.EDriveMain.NonCharging.Normal.Mode2.EWP1.Level4 [order 1] : [PRC]
                  (junction 377) -> (junction 375)
                  (junction 375) -> ON.Normal.EDrive.EDriveMain.NonCharging.Normal.Mode2.EWP1.Level2 [order 1] : [CabinMode>=8&&ACSubMode==2]
                  (junction 375) -> ON.Normal.EDrive.EDriveMain.NonCharging.Normal.Mode2.EWP1.Level3 [order 2]
                  ON.Normal.EDrive.EDriveMain.NonCharging.Normal.Mode2.EWP1.Level2 -> ON.Normal.EDrive.EDriveMain.NonCharging.Normal.Mode2.EWP1.Level3 [order 2] : [CabinMode<8||ACSubMode!=2]
                  ON.Normal.EDrive.EDriveMain.NonCharging.Normal.Mode2.EWP1.Level3 -> ON.Normal.EDrive.EDriveMain.NonCharging.Normal.Mode2.EWP1.Level2 [order 2] : [CabinMode>=8&&ACSubMode==2]
                state ACPressureLow2 [parallel]
                  settings: executionOrder=3
                  state LV1
                    en:ACLPLV=uint8(1);
                  state LV2
                    en:ACLPLV=uint8(2);
                  state LV3
                    en:ACLPLV=uint8(3);
                  state LV4
                    en:ACLPLV=uint8(4);
                  state LV5
                    en:ACLPLV=uint8(5);
                  (default) -> (junction 403)
                  (junction 403) -> ON.Normal.EDrive.EDriveMain.NonCharging.Normal.Mode2.ACPressureLow2.LV1 [order 1] : [CabinMode<=2]
                  (junction 403) -> (junction 404) [order 2]
                  ON.Normal.EDrive.EDriveMain.NonCharging.Normal.Mode2.ACPressureLow2.LV1 -> ON.Normal.EDrive.EDriveMain.NonCharging.Normal.Mode2.ACPressureLow2.LV2 : [CabinMode>2]
                  ON.Normal.EDrive.EDriveMain.NonCharging.Normal.Mode2.ACPressureLow2.LV2 -> ON.Normal.EDrive.EDriveMain.NonCharging.Normal.Mode2.ACPressureLow2.LV1 [order 2] : [CabinMode<=2]
                  (junction 404) -> ON.Normal.EDrive.EDriveMain.NonCharging.Normal.Mode2.ACPressureLow2.LV2 [order 1] : [CabinMode>2]
                  (junction 404) -> (junction 405) [order 2]
                  ON.Normal.EDrive.EDriveMain.NonCharging.Normal.Mode2.ACPressureLow2.LV2 -> ON.Normal.EDrive.EDriveMain.NonCharging.Normal.Mode2.ACPressureLow2.LV3 [order 1] : [ACLP<KTHC_P2MinLo_kPa]
                  ON.Normal.EDrive.EDriveMain.NonCharging.Normal.Mode2.ACPressureLow2.LV3 -> ON.Normal.EDrive.EDriveMain.NonCharging.Normal.Mode2.ACPressureLow2.LV2 [order 2] : [ACLP>KTHC_P3MaxLo_kPa]
                  (junction 405) -> ON.Normal.EDrive.EDriveMain.NonCharging.Normal.Mode2.ACPressureLow2.LV3 [order 1] : [ACLP>KTHC_P4MaxLo_kPa]
                  (junction 405) -> (junction 406) [order 2]
                  ON.Normal.EDrive.EDriveMain.NonCharging.Normal.Mode2.ACPressureLow2.LV3 -> ON.Normal.EDrive.EDriveMain.NonCharging.Normal.Mode2.ACPressureLow2.LV4 [order 1] : [ACLP<KTHC_P3MinLo_kPa]
                  ON.Normal.EDrive.EDriveMain.NonCharging.Normal.Mode2.ACPressureLow2.LV4 -> ON.Normal.EDrive.EDriveMain.NonCharging.Normal.Mode2.ACPressureLow2.LV3 [order 2] : [ACLP>KTHC_P4MaxLo_kPa]
                  (junction 406) -> ON.Normal.EDrive.EDriveMain.NonCharging.Normal.Mode2.ACPressureLow2.LV4 [order 1] : [ACLP>KTHC_P5MaxLo_kPa]
                  (junction 406) -> (junction 407) [order 2]
                  ON.Normal.EDrive.EDriveMain.NonCharging.Normal.Mode2.ACPressureLow2.LV4 -> ON.Normal.EDrive.EDriveMain.NonCharging.Normal.Mode2.ACPressureLow2.LV5 [order 1] : [ACLP<KTHC_P4MinLo_kPa]
                  ON.Normal.EDrive.EDriveMain.NonCharging.Normal.Mode2.ACPressureLow2.LV5 -> ON.Normal.EDrive.EDriveMain.NonCharging.Normal.Mode2.ACPressureLow2.LV4 : [ACLP>KTHC_P5MaxLo_kPa]
                  (junction 407) -> ON.Normal.EDrive.EDriveMain.NonCharging.Normal.Mode2.ACPressureLow2.LV5
                state Fagsfan [parallel]
                  settings: executionOrder=4
                  state AGS_FAN_FLAG_OFF
                    en:Fagsfan=false;
                  state AGS_FAN_FLAG_ON
                    en:Fagsfan=true;
                  (default) -> (junction 473)
                  (junction 473) -> AGS_FAN_FLAG_OFF [order 1] : [Tsat_low2>=Tamb]
                  (junction 473) -> (junction 474) [order 2]
                  AGS_FAN_FLAG_ON -> AGS_FAN_FLAG_OFF : [Tsat_low2>=Tamb&&!PRC]
                  AGS_FAN_FLAG_OFF -> AGS_FAN_FLAG_ON : [Tsat_low2<Tamb-KTHC_DTambSat5_C||PRC]
                  (junction 474) -> AGS_FAN_FLAG_ON
                state EWP2 [parallel]
                  settings: executionOrder=7
                  state Level4
                    en:EWP2=4;
                  state Level2
                    en:EWP2=2;
                  state Level3
                    en:EWP2=3;
                  (default) -> (junction 1277)
                  (junction 1277) -> ON.Normal.EDrive.EDriveMain.NonCharging.Normal.Mode2.EWP2.Level4 [order 1] : [PRC]
                  (junction 1277) -> (junction 1278) [order 2]
                  ON.Normal.EDrive.EDriveMain.NonCharging.Normal.Mode2.EWP2.Level4 -> (junction 1279) : [!PRC]
                  ON.Normal.EDrive.EDriveMain.NonCharging.Normal.Mode2.EWP2.Level2 -> ON.Normal.EDrive.EDriveMain.NonCharging.Normal.Mode2.EWP2.Level4 [order 1] : [PRC]
                  ON.Normal.EDrive.EDriveMain.NonCharging.Normal.Mode2.EWP2.Level3 -> ON.Normal.EDrive.EDriveMain.NonCharging.Normal.Mode2.EWP2.Level4 [order 1] : [PRC]
                  (junction 1278) -> (junction 1279)
                  (junction 1279) -> ON.Normal.EDrive.EDriveMain.NonCharging.Normal.Mode2.EWP2.Level2 [order 1] : [CabinMode>=8&&ACSubMode==2]
                  (junction 1279) -> ON.Normal.EDrive.EDriveMain.NonCharging.Normal.Mode2.EWP2.Level3 [order 2]
                  ON.Normal.EDrive.EDriveMain.NonCharging.Normal.Mode2.EWP2.Level2 -> ON.Normal.EDrive.EDriveMain.NonCharging.Normal.Mode2.EWP2.Level3 [order 2] : [CabinMode<8||ACSubMode!=2]
                  ON.Normal.EDrive.EDriveMain.NonCharging.Normal.Mode2.EWP2.Level3 -> ON.Normal.EDrive.EDriveMain.NonCharging.Normal.Mode2.EWP2.Level2 [order 2] : [CabinMode>=8&&ACSubMode==2]
                state TWV [parallel]
                  settings: executionOrder=2
                  state PRC_OFF
                    en:PRC=false;
                    TWV=0;
                  state PRC_ON
                    en:PRC=true;
                    TWV=KTHC_TWVRcolPos_pct;
                  (default) -> PRC_OFF
                  PRC_OFF -> PRC_ON : [Motor_In_Temp>KTHC_TwRcolOn_C || BatteryMode==2]
                  PRC_ON -> PRC_OFF : [Motor_In_Temp<KTHC_TwRcolOff_C && BatteryMode!=2]
                state FAN [parallel]
                  settings: executionOrder=5
                  state S1
                    en:FAN=1;
                  state S2
                    en:FAN=4;
                  note: AC Dehumidty Mode=1
                  state S3
                    en:FAN=1;
                  note: HeatingMode=2.2
                  note: HeatingMode=1.2
                  state S4
                    en:FAN=2;
                  note: HeatingMode=1.1 or 2.1
                  state S5
                    en:FAN=ACLPLV;
                  state S6
                    en:FAN=3;
                  (default) -> (junction 484)
                  ON.Normal.EDrive.EDriveMain.NonCharging.Normal.Mode2.FAN -> (junction 484)
                  (junction 484) -> ON.Normal.EDrive.EDriveMain.NonCharging.Normal.Mode2.FAN.S1 [order 1] : [!Fagsfan||!Ffan]
                  (junction 484) -> (junction 485) [order 2]
                  (junction 485) -> ON.Normal.EDrive.EDriveMain.NonCharging.Normal.Mode2.FAN.S2 [order 1] : [PRC]
                  (junction 485) -> (junction 486) [order 2]
                  (junction 486) -> ON.Normal.EDrive.EDriveMain.NonCharging.Normal.Mode2.FAN.S3 [order 1] : [CabinMode==4]
                  (junction 486) -> (junction 1255) [order 2]
                  (junction 1255) -> ON.Normal.EDrive.EDriveMain.NonCharging.Normal.Mode2.FAN.S3 [order 1] : [CabinMode==9&&ACSubMode==2]
                  (junction 1255) -> (junction 1550) [order 2]
                  (junction 1550) -> ON.Normal.EDrive.EDriveMain.NonCharging.Normal.Mode2.FAN.S3 [order 1] : [!AC&&BatteryMode==4]
                  (junction 1550) -> (junction 1259) [order 2]
                  (junction 1259) -> ON.Normal.EDrive.EDriveMain.NonCharging.Normal.Mode2.FAN.S4 [order 1] : [CabinMode==8&&ACSubMode==2]
                  (junction 1259) -> (junction 489) [order 2]
                  (junction 489) -> ON.Normal.EDrive.EDriveMain.NonCharging.Normal.Mode2.FAN.S5 [order 1] : [CabinMode>=8]
                  (junction 489) -> ON.Normal.EDrive.EDriveMain.NonCharging.Normal.Mode2.FAN.S6 [order 2]
                state AGS [parallel]
                  settings: executionOrder=6
                  state S1
                    en:AGS=1;
                  state S2
                    en:AGS=5;
                  state S3
                    en:AGS=4;
                  note: AC Dehunidty Mode=1
                  state S4
                    en:AGS=1;
                  note: HeatingMode=2.2
                  note: HeatingMode=1.2
                  state S5
                    en:AGS=2;
                  note: HeatingMode=1.1 or 2.1
                  state S6
                    en:AGS=ACLPLV;
                  state S7
                    en:AGS=3;
                  (default) -> (junction 539)
                  ON.Normal.EDrive.EDriveMain.NonCharging.Normal.Mode2.AGS -> (junction 539)
                  (junction 539) -> ON.Normal.EDrive.EDriveMain.NonCharging.Normal.Mode2.AGS.S1 [order 1] : [Fags==3||!Fagsfan]
                  (junction 539) -> (junction 540) [order 2]
                  (junction 540) -> ON.Normal.EDrive.EDriveMain.NonCharging.Normal.Mode2.AGS.S2 [order 1] : [Fags==1&&(CabinMode!=9||....
                      | ACSubMode!=2)&&....
                      | CabinMode!=4&&....
                      | (AC||BatteryMode!=4)]
                  (junction 540) -> (junction 541) [order 2]
                  (junction 541) -> ON.Normal.EDrive.EDriveMain.NonCharging.Normal.Mode2.AGS.S3 [order 1] : [PRC]
                  (junction 541) -> (junction 542) [order 2]
                  (junction 542) -> ON.Normal.EDrive.EDriveMain.NonCharging.Normal.Mode2.AGS.S4 [order 1] : [CabinMode==4]
                  (junction 542) -> (junction 545) [order 2]
                  (junction 545) -> ON.Normal.EDrive.EDriveMain.NonCharging.Normal.Mode2.AGS.S4 [order 1] : [CabinMode==9&&ACSubMode==2]
                  (junction 545) -> (junction 1558) [order 2]
                  (junction 1558) -> ON.Normal.EDrive.EDriveMain.NonCharging.Normal.Mode2.AGS.S4 [order 1] : [!AC&&BatteryMode==4]
                  (junction 1558) -> (junction 1297) [order 2]
                  (junction 1297) -> ON.Normal.EDrive.EDriveMain.NonCharging.Normal.Mode2.AGS.S5 [order 1] : [CabinMode==8&&ACSubMode==2]
                  (junction 1297) -> (junction 1300) [order 2]
                  (junction 1300) -> ON.Normal.EDrive.EDriveMain.NonCharging.Normal.Mode2.AGS.S6 [order 1] : [CabinMode>=8]
                  (junction 1300) -> S7 [order 2]
              (junction 596) -> (junction 595) [order 1] : [RequestTWV||ReqWasteHeatRecovery]
              (junction 596) -> ON.Normal.EDrive.EDriveMain.NonCharging.Normal.Mode1 [order 2]
              (junction 595) -> ON.Normal.EDrive.EDriveMain.NonCharging.Normal.Mode2
              ON.Normal.EDrive.EDriveMain.NonCharging.Normal.Mode1 -> ON.Normal.EDrive.EDriveMain.NonCharging.Normal.Mode2 : [RequestTWV||ReqWasteHeatRecovery]
              ON.Normal.EDrive.EDriveMain.NonCharging.Normal.Mode2 -> ON.Normal.EDrive.EDriveMain.NonCharging.Normal.Mode1 : [!RequestTWV&&!ReqWasteHeatRecovery]
              (junction 2350) -> ON.Normal.EDrive.EDriveMain.NonCharging.Normal.Mode2
              (junction 2352) -> ON.Normal.EDrive.EDriveMain.NonCharging.Normal.Mode1
              (junction 2349) -> (junction 2352) [order 2] : [NormalMode == 1]
              (junction 2349) -> (junction 2350) [order 1] : [NormalMode == 2]
            state Deicing
              en:EDriveMode=uint8(3);TWV=100;
              state Normal
                en:EWP1=2;
                EWP2=2;
                FAN=1;
                AGS=1;
              state OverHeat
                en:EWP1=4;
                EWP2=4;
                FAN=4;
                AGS=4;
              (default) -> (junction 2141)
              (junction 2141) -> ON.Normal.EDrive.EDriveMain.NonCharging.Deicing.Normal [order 2]
              (junction 2141) -> OverHeat [order 1] : [Motor_In_Temp>KTHC_TwOhtOn_C]
              ON.Normal.EDrive.EDriveMain.NonCharging.Deicing.Normal -> OverHeat : [Motor_In_Temp>KTHC_TwOhtOn_C]
              OverHeat -> ON.Normal.EDrive.EDriveMain.NonCharging.Deicing.Normal : [Motor_In_Temp<KTHC_TwOhtOff_C]
            (default) -> (junction 596)
            ON.Normal.EDrive.EDriveMain.NonCharging.Deicing -> (junction 2349) : [DeiceModeReq==0]
            ON.Normal.EDrive.EDriveMain.NonCharging.Normal -> ON.Normal.EDrive.EDriveMain.NonCharging.Deicing : [DeiceModeReq==1]
          state Charging
            en:
            EDriveMode=4;
            TWV=0;
            EWP1=8;
            EWP2=8;
            FAN=1;
            AGS=1;
          (default) -> NonCharging
          NonCharging -> Charging : [BatteryMode==7]
          Charging -> NonCharging : [BatteryMode!=7]
        state Ffan [parallel]
          settings: executionOrder=1
          state LowSpeed
            en:Ffan=true;
          state HighSpeed
            en:Ffan=false;
          (default) -> ON.Normal.EDrive.Ffan.LowSpeed
          ON.Normal.EDrive.Ffan.LowSpeed -> ON.Normal.EDrive.Ffan.HighSpeed : [VehSpeed>KTHC_VehSdFanOff_kph]
          ON.Normal.EDrive.Ffan.HighSpeed -> ON.Normal.EDrive.Ffan.LowSpeed : [VehSpeed<KTHC_VehSdFanOn_kph]
        state Fags [parallel]
          settings: executionOrder=2
          state ON
            state HighSpeed
              en:Fags=2;
            state LowSpeed
              en:Fags=1;
            (default) -> ON.Normal.EDrive.Fags.ON.LowSpeed
            ON.Normal.EDrive.Fags.ON.LowSpeed -> ON.Normal.EDrive.Fags.ON.HighSpeed : [VehSpeed>KTHC_VehSdAGSCtrl_kph]
            ON.Normal.EDrive.Fags.ON.HighSpeed -> ON.Normal.EDrive.Fags.ON.LowSpeed : [VehSpeed<KTHC_VehSdAGS100_kph]
          state OFF
            en:Fags=3;
          (default) -> ON.Normal.EDrive.Fags.OFF
          ON.Normal.EDrive.Fags.ON -> ON.Normal.EDrive.Fags.OFF : [PwrSta==0||....
              | (VSCP_AGSCloseSta_flg==1&&....
              | ShiftGearPosn==4)]
          ON.Normal.EDrive.Fags.OFF -> ON.Normal.EDrive.Fags.ON : [PwrSta>0&&....
              | (VSCP_AGSCloseSta_flg==0||....
              | ShiftGearPosn!=4)]
      state DeiceDetect [parallel]
        settings: executionOrder=1
        state Comp [parallel]
          settings: executionOrder=5
          state CompOFF
          state CompON
          (default) -> (junction 2519)
          (junction 2519) -> ON.Normal.DeiceDetect.Comp.CompOFF [order 1] : [CompSpd==0]
          (junction 2519) -> ON.Normal.DeiceDetect.Comp.CompON [order 2]
          ON.Normal.DeiceDetect.Comp.CompON -> ON.Normal.DeiceDetect.Comp.CompOFF : [CompSpd==0]
          ON.Normal.DeiceDetect.Comp.CompOFF -> (junction 2524) : [CompSpd>=800]
          (junction 2524) -> ON.Normal.DeiceDetect.Comp.CompON [order 1] : [CabinMode==10]
          (junction 2524) -> (junction 2526) [order 2]
          (junction 2526) -> ON.Normal.DeiceDetect.Comp.CompON : {DeiceDetReset=1;}
        state DriverDeice [parallel]
          settings: executionOrder=2
          (default) -> (junction 2197) : {DriveDeice=0;}
          DriverDeice -> (junction 2197) [order 1] : [hasChanged(DeiceModeReq)&&....
              | DeiceModeReq==0]
          (junction 2197) -> (junction 2291)
          DriverDeice -> (junction 2291) [order 2] : [DeiceDetReset]
          (junction 2291) -> (junction 1982) : {FirstDet=1;AvgCnt=0;dy=0;Tsum=0;DataCnt=0;DeiceDetReset=0;}
          DriverDeice -> (junction 1982) [order 3] : [DeiceModeReq==0&&...
              | !(Tamb<=KTHC_TambHPmin_C&&....
              | CabinMode==9&&ACSubMode==2)]
          (junction 1982) -> (junction 1983) : {DataCnt=DataCnt+1;Tsum=Tsum+Tamb-Tsat_low2;}
          (junction 1983) -> (junction 1984) [order 1] : [!FirstDet&&DataCnt==KTHC_tb_K]
          (junction 1983) -> (junction 1987) [order 2]
          (junction 1984) -> (junction 1985)
          (junction 1987) -> (junction 1985) [order 1] : [DataCnt==KTHC_ta_K]
          (junction 1987) -> (junction 1986) [order 2]
          (junction 1985) -> (junction 1988) : {Tavg1=Tavg2;....
              | Tavg2=Tavg3;....
              | Tavg3=Tavg4;....
              | Tavg4=Tavg5;
              | Tavg5=Tsum/DataCnt;
              | Tsum=0;
              | DataCnt=0;
              | FirstDet=0;}
          (junction 1986) -> (junction 2201) [order 2]
          (junction 1988) -> (junction 1986) [order 1] : [AvgCnt==6]{dy=Tavg5-Tavg1;}
          (junction 1988) -> (junction 1989) [order 2] : {AvgCnt=AvgCnt+1;}
          (junction 1986) -> (junction 1990) [order 1] : [Tamb<KTHC_TDeice2_C&&....
              | ChrgPlugSta==0]
          (junction 1990) -> (junction 1991) [order 1] : [dy>dAy]
          (junction 1990) -> (junction 1992) [order 2]
          (junction 1991) -> (junction 1994)
          (junction 1992) -> (junction 1994) : [Tamb>KTHC_TambHPmin_C&&....
              | CabinMode==9&&ACSubMode==2]
          (junction 1994) -> (junction 1993) : {DriveDeice=1;}
        state ChargeDeice [parallel]
          settings: executionOrder=3
          (default) -> (junction 1977) : {FirstCharDeice=1;}
          ChargeDeice -> (junction 1977)
          (junction 1977) -> (junction 2019) [order 1] : [FirstCharDeice==0]
          (junction 1977) -> (junction 2028) [order 2]
          (junction 2019) -> (junction 2033)
          (junction 2028) -> (junction 2033) [order 1] : [ChrgPlugSta==0]
          (junction 2028) -> (junction 2029) [order 2]
          (junction 2033) -> (junction 2035)
          (junction 2029) -> (junction 2035) [order 1] : [DeiceCycle==0]
          (junction 2029) -> (junction 2012) [order 2]
          (junction 2035) -> (junction 2030)
          (junction 2012) -> (junction 2030) [order 1] : [Tamb>=KTHC_TDeice1_C]
          (junction 2012) -> (junction 2022) [order 2] : {ChargeDeice=1;FirstCharDeice=0;}
          (junction 2030) -> (junction 2023) : {ChargeDeice=0;}
        state Cabin92to91 [parallel]
          settings: executionOrder=1
          state CabinModenot9
          state CabinMode91
          state CabinMode92
          (default) -> CabinModenot9
          CabinMode91 -> CabinModenot9 [order 1] : [CabinMode!=9]
          CabinModenot9 -> (junction 2306) : [CabinMode==9]
          (junction 2306) -> CabinMode91 [order 2]
          (junction 2306) -> CabinMode92 [order 1] : [ACSubMode==2]
          CabinMode91 -> CabinMode92 [order 2] : [ACSubMode==2]
          CabinMode92 -> CabinMode91 [order 2] : [ACSubMode==1]....
              | {DeiceDetReset=1;}
          CabinMode92 -> CabinModenot9 [order 1] : [CabinMode!=9]
        state DeiceReq [parallel]
          settings: executionOrder=4
          state NoReq
            en:DeiceModeReq=0;
            DeiceCycle=1;
          state Req
            en:DeiceModeReq=1;
            DeiceCycle=0;
            DriveDeice=0;
          state WaitForRestart
            DeiceModeReq=0;
          (default) -> NoReq
          NoReq -> Req : [DriveDeice==1||ChargeDeice==1]
          WaitForRestart -> NoReq : [after(KTHC_DeiceCycTime_K,tick)]
          Req -> WaitForRestart : [(after(200,tick)&&ACHP>KTHC_PDeiceMax_kPa)||....
              | after(KTHC_TimeDeiceMax_K,tick)]
    (default) -> ON.Normal
    ON.Normal -> WaterFill : [WaterFillReq>0]
    WaterFill -> ON.Normal : [WaterFillReq==0]
  (default) -> OFF
  OFF -> ON : [VPMM_SysPwrSta_enum!=0&&....
      | VPMM_SysPwrSta_enum!=3&&....
      | VPMM_SysPwrSta_enum!=6&&....
      | VPMM_SysPwrSta_enum!=7]
  ON -> OFF : [VPMM_SysPwrSta_enum==0||....
      | VPMM_SysPwrSta_enum==3||....
      | VPMM_SysPwrSta_enum==6||....
      | VPMM_SysPwrSta_enum==7]
  data: ACMax input; Bat_In_Temp input; CompSpd input; Motor_In_Temp input; Motor_Out_Temp input; PT_Low_P2 input; PwrSta input; TBMax input; TBMin input; TFrMCU input; TFrTM input; TRrMCU input; TRrTM input; Tamb input; Tdcdc input; Tevap input; Tincar input; Tobc input; Tsat_low2 input; VehSpeed input; sigSetTempZon1St input; AGS output double; FAN output double; FrWPTCHeatPwr output double; BattPump3 output uint8; BlowerPID output double; CompPID output uint8; CompSet output double; EWP1 output double; EWP2 output double; EXV2PIDMode output uint8; FWV output boolean; SOTXV output boolean; TWV output single; APTCPID output uint8; ACHPLV local double; ACLPLV local double; ACSubMode output uint8; BatteryLV local double; BatteryMode output uint8; CabinCompReq local boolean; CabinMode output uint8; DCDCLV local double; EDriveLV2 local uint8; Fags local uint8; Fagsfan local boolean; Ffan local boolean; FrMCULV local double; FrTMLV local double; OBCLV local double; PRC local boolean; ReqWasteHeatRecovery local boolean; RequestCOMP local boolean; RequestTWV local boolean; RrMCULV local double; RrTMLV local double; TincarPos local boolean; WaterCompReq local boolean; AC input; sigSetTempZon1StC input; ACMaxReq local boolean; ACHP input; ACLP input double; PT_High_T input; EDriveMode output double; APTCQ input double; VSCP_AGSCloseSta_flg input; ShiftGearPosn input; EDriveLV1 local uint8; EDriveLV3 local uint8; EDriveLV4 local uint8; ACD3Lv local double; ChrgPlugSta input; Timehu1 input; Timehu2 input; Tice input; Tdeice input; EvapDefog local boolean; DfrstReq input; FanMax local boolean =false; WaterFillReq input; APTCQminD input; KTHC_T1MaxBC_C input; KTHC_T2MinBC_C input; KTHC_T2MaxBC_C input; KTHC_T3MinBC_C input; KTHC_T3MaxBC_C input; KTHC_T4MinBC_C input; KTHC_T4MaxBC_C input; KTHC_T5MinBC_C input; KTHC_T1MaxCCU_C input; KTHC_T2MinCCU_C input; KTHC_T2MaxCCU_C input; KTHC_T3MinCCU_C input; KTHC_T3MaxCCU_C input; KTHC_T4MinCCU_C input; KTHC_T4MaxCCU_C input; KTHC_T5MinCCU_C input; KTHC_T1MaxMCU_C input; KTHC_T2MinMCU_C input; KTHC_T2MaxMCU_C input; KTHC_T3MinMCU_C input; KTHC_T3MaxMCU_C input; KTHC_T4MinMCU_C input; KTHC_T4MaxMCU_C input; KTHC_T5MinMCU_C input; KTHC_T1MaxMT_C input; KTHC_T2MinMT_C input; KTHC_T2MaxMT_C input; KTHC_T3MinMT_C input; KTHC_T3MaxMT_C input; KTHC_T4MinMT_C input; KTHC_T4MaxMT_C input; KTHC_T5MinMT_C input; KTHC_P2MaxHi_kPa input; KTHC_P3MinHi_kPa input; KTHC_P3MaxHi_kPa input; KTHC_P4MinHi_kPa input; KTHC_P4MaxHi_kPa input; KTHC_P5MinHi_kPa input; KTHC_P2MinLo_kPa input; KTHC_P3MaxLo_kPa input; KTHC_P3MinLo_kPa input; KTHC_P4MaxLo_kPa input; KTHC_P4MinLo_kPa input; KTHC_P5MaxLo_kPa input; KTHC_TWVRcolPos_pct input; KTHC_TwRcolOn_C input; KTHC_TwRcolOff_C input; KTHC_DTambSat_C input; KTHC_VehSdFanOn_kph input; KTHC_VehSdFanOff_kph input; KTHC_VehSdAGS100_kph input; KTHC_VehSdAGSCtrl_kph input; KTHC_T1MinBH_C input; KTHC_T2MaxBH_C input; KTHC_T2MinBH_C input; KTHC_T3MaxBH_C input; KTHC_T3MinBH_C input; KTHC_T4MaxBH_C input; KTHC_T4MinBH_C input; KTHC_T5MaxBH_C input; T2MaxBAH input; T2MinBAH input; T3MaxBAH input; T3MinBAH input; T4MaxBAH input; LevelWPTCBAH1 input; LevelWPTCBAH2 input; LevelWPTCBAH3 input; LevelWPTCBAH4 input; KTHC_TWinmax_C input; KTHC_TWinmin_C input; KTHC_DTwBMoin1_C input; KTHC_DTwBMoin2_C input; KTHC_DTwBBin_C input; KTHC_CompSpdmax_rpm input; KTHC_TBPmax_C input; KTHC_TBPmin_C input; KTHC_T3winSetpointBC_C input; KTHC_Timewcd_K input; KTHC_CompSpdmin_rpm input; KTHC_Plow2Setpoint_kPa input; KTHC_DTh1_C input; KTHC_Tambset_C input; KTHC_Twmset_C input; KTHC_APTCQminRe_W input; KTHC_CompSpdmid_rpm input; KTHC_PhiDehum_kPa input; KTHC_ThiDehum_C input; KTHC_TimeD_K input; KTHC_Tdefog_C input; KTHC_Tdeheat1_C input; KTHC_Tdeheat2_C input; KTHC_DehumidityEN_flg input; dAy input; Bat_Out_Temp input; KTHC_CompMaxDeice_rpm input; KTHC_CompMinDeice_rpm input; KTHC_DeiceCycTime_K input; KTHC_PDeiceMax_kPa input; T1MinBAH input; KTHC_TDeice1_C input; KTHC_TDeice2_C input; KTHC_TambHPmin_C input; KTHC_Time0_K input; KTHC_TimeDeiceMax_K input; KTHC_TwOhtOff_C input; KTHC_TwOhtOn_C input; KTHC_aDeice_K input; KTHC_bDeice_K input; KTHC_ta_K input; KTHC_tb_K input; AvgCnt local uint8; ChargeDeice local boolean; DataCnt local uint16; DeiceCycle local boolean; DeiceModeReq local boolean; DriveDeice local boolean; FirstCharDeice local boolean; FirstDet local boolean; Tavg1 local double; Tavg2 local double; Tavg3 local double; Tavg4 local double; Tavg5 local double; Tsum local double; KTHC_T1MaxLLC_C input; KTHC_T2MinLLC_C input; KTHC_T2MaxLLC_C input; KTHC_T3MinLLC_C input; KTHC_T3MaxLLC_C input; KTHC_T4MinLLC_C input; KTHC_T4MaxLLC_C input; KTHC_T5MinLLC_C input; Fr_LLCTemp input; Rr_LLCTemp input; FrLLCLV local double; RrLLCLV local double; dy output double; PET input; EACProtectEnable input; ForceComp local boolean; KTHC_TDcChgBC_C input; ErrCompForceOFF input; KTHC_CompSpdmaxBC_rpm input; Tamb_Err input; DeiceDetReset local boolean; KTHC_DTcabin_C input; KTHC_DTreturn1_C input; KTHC_DTreturn_C input; KTHC_DTcabin1_C input; KTHC_DTcabin2_C input; KTHC_DTreturn3_C input; KTHC_DTimeCD_K input; KTHC_DTambSat1_C input; KTHC_DTambSat2_C input; CabinCompReqCancel local boolean; KTHC_APTCQMaxC_W input; KTHC_DTreturn2_C input; KTHC_DTcabin3_C input; KTHC_DTcabin4_C input; KTHC_DTcabin5_C input; KTHC_DTcabin6_C input; KTHC_DTimeCD1_K input; KTHC_DTimeCD2_K input; KTHC_TambACmode1_C input; KTHC_TambACmode2_C input; KTHC_TambACmode3_C input; KTHC_TambACmode4_C input; KTHC_DTcabin7_C input; NormalMode local uint8; PumpONmode local uint8; ACSubModeLAST local uint8; KTHC_DTcabin9_C input; KTHC_DTcabin10_C input; KTHC_DTreturn6_C input; KTHC_DTambSat5_C input; FCool local uint8; KTHC_APTCQminRe1_W input; KTHC_DTCabin11_C input; KTHC_TambSetLow_C input; KTHC_Tcoolmin_C input; KTHC_TimeRe1_sec input; KTHC_TimeRe2_sec input; KTHC_Trecymin_C input; KTHC_WoWPTC_flg input; BatDcCharge local double; KTHC_DTreturn7_C input; KTHC_DTambsat3_C input; KTHC_TambACmode5_C input; KTHC_TambACmode6_C input; KTHC_CompSpdmid1_rpm input; KTHC_CompSpdmid2_rpm input; KTHC_CompSpdmid3_rpm input; KTHC_DTcabin12_C input; KTHC_CompSpdmaxBC1_rpm input; KTHC_DTambsat4_C input; KTHC_TambACmode7_C input; VINP_HVBattSOCDis_pct input single; VINP_IVIWPTCSWSta_flg input boolean; PreWPTC local boolean; VTHC_FDCTHCMPreWPTCHeatSta_enum output uint8; KTHC_DTwBMoin3_C input; TambMax local single; TambMin local single; KTHC_ForceLeaveCool_C input; KTHC_ForceLeaveHeat_C input; CabinModeReset local boolean; KTHC_BatCoolT_cnt input; VPMM_SysPwrSta_enum input uint8
  events: eWPTCSW local FUNCTION_CALL_EVENT
